simulink model "model"  (R2014a)
(part 6 of 6)

  _CN_235143897_220000_CN_21239912_220000/LConn1 -- T_235143897__SP_AusNet_Brooklyn_Terminal_Station/LConn1 -- _CN_235143897_220000_CN_384601555_220000/LConn1 -- _CN_235143897_220000_CN_243897689_220000/LConn1
  _CN_235143897_220000_CN_21239912_220000/LConn2 -- T_235143897__SP_AusNet_Brooklyn_Terminal_Station/LConn2 -- _CN_235143897_220000_CN_384601555_220000/LConn2 -- _CN_235143897_220000_CN_243897689_220000/LConn2
  _CN_235143897_220000_CN_21239912_220000/LConn3 -- T_235143897__SP_AusNet_Brooklyn_Terminal_Station/LConn3 -- _CN_235143897_220000_CN_384601555_220000/LConn3 -- _CN_235143897_220000_CN_243897689_220000/LConn3 -- bus266/LConn1
  _CN_235143897_220000_CN_21239912_220000/RConn1 -- T_21239912__AusNet_Keilor_Terminal_Station/RConn1 -- _CN_23718970_220000_CN_21239912_220000/LConn1 -- _CN_21239912_220000_CN_208198646_220000/LConn1 -- L_21239912/LConn1 -- _CN_244141232_220000_CN_21239912_220000/LConn1
  _CN_235143897_220000_CN_21239912_220000/RConn2 -- T_21239912__AusNet_Keilor_Terminal_Station/RConn2 -- _CN_23718970_220000_CN_21239912_220000/LConn2 -- _CN_21239912_220000_CN_208198646_220000/LConn2 -- L_21239912/LConn2 -- _CN_244141232_220000_CN_21239912_220000/LConn2
  _CN_235143897_220000_CN_21239912_220000/RConn3 -- T_21239912__AusNet_Keilor_Terminal_Station/RConn3 -- _CN_23718970_220000_CN_21239912_220000/LConn3 -- _CN_21239912_220000_CN_208198646_220000/LConn3 -- L_21239912/LConn3 -- bus267/LConn1 -- _CN_244141232_220000_CN_21239912_220000/LConn3
  _CN_235143897_220000_CN_384601555_220000/RConn1 -- T_384601555__AusNet_Fishermans_Bend_Terminal_Station/LConn1 -- _CN_384601555_220000_CN_208198646_220000/LConn1
  _CN_235143897_220000_CN_384601555_220000/RConn2 -- T_384601555__AusNet_Fishermans_Bend_Terminal_Station/LConn2 -- _CN_384601555_220000_CN_208198646_220000/LConn2
  _CN_235143897_220000_CN_384601555_220000/RConn3 -- T_384601555__AusNet_Fishermans_Bend_Terminal_Station/LConn3 -- _CN_384601555_220000_CN_208198646_220000/LConn3 -- bus268/LConn1
  G_243897689_Ecogen_Newport_Power_Station/RConn1 -- _CN_235143897_220000_CN_243897689_220000/RConn1
  G_243897689_Ecogen_Newport_Power_Station/RConn2 -- _CN_235143897_220000_CN_243897689_220000/RConn2
  _CN_235143897_220000_CN_243897689_220000/RConn3 -- G_243897689_Ecogen_Newport_Power_Station/RConn3 -- bus269/LConn1
  T_23298443__/LConn1 -- _CN_23298443_220000_CN_87324834_220000/LConn1
  T_23298443__/LConn2 -- _CN_23298443_220000_CN_87324834_220000/LConn2
  _CN_23298443_220000_CN_87324834_220000/LConn3 -- T_23298443__/LConn3 -- bus270/LConn1
  _CN_23298443_220000_CN_87324834_220000/RConn1 -- G_87324834_Liapootah_Power_Station/RConn1 -- _CN_87325631_220000_CN_87324834_220000/LConn1
  _CN_23298443_220000_CN_87324834_220000/RConn2 -- G_87324834_Liapootah_Power_Station/RConn2 -- _CN_87325631_220000_CN_87324834_220000/LConn2
  _CN_23298443_220000_CN_87324834_220000/RConn3 -- G_87324834_Liapootah_Power_Station/RConn3 -- _CN_87325631_220000_CN_87324834_220000/LConn3 -- bus271/LConn1
  T_167791635__Burnie_Substation/LConn1 -- _CN_167791635_220000_CN_88191017_220000/LConn1
  T_167791635__Burnie_Substation/LConn2 -- _CN_167791635_220000_CN_88191017_220000/LConn2
  _CN_167791635_220000_CN_88191017_220000/LConn3 -- T_167791635__Burnie_Substation/LConn3 -- bus272/LConn1
  _CN_167791635_220000_CN_88191017_220000/RConn1 -- T_88191017__/LConn1 -- _CN_88191017_220000_CN_174441055_220000/RConn1
  _CN_167791635_220000_CN_88191017_220000/RConn2 -- T_88191017__/LConn2 -- _CN_88191017_220000_CN_174441055_220000/RConn2
  _CN_167791635_220000_CN_88191017_220000/RConn3 -- T_88191017__/LConn3 -- _CN_88191017_220000_CN_174441055_220000/RConn3 -- bus273/LConn1
  _CN_24054804_220000_CN_28225387_220000/LConn1 -- T_24054804__SP_AusNet_Rowville_Terminal_Station/RConn1 -- _CN_24054804_220000_CN_30837800_220000/LConn1 -- _CN_24054804_220000_CN_134534513_220000/LConn1 -- L_24054804/LConn1 -- _CN_24054804_220000_CN_239972088_220000/LConn1
  _CN_24054804_220000_CN_28225387_220000/LConn2 -- T_24054804__SP_AusNet_Rowville_Terminal_Station/RConn2 -- _CN_24054804_220000_CN_30837800_220000/LConn2 -- _CN_24054804_220000_CN_134534513_220000/LConn2 -- L_24054804/LConn2 -- _CN_24054804_220000_CN_239972088_220000/LConn2
  _CN_24054804_220000_CN_28225387_220000/LConn3 -- T_24054804__SP_AusNet_Rowville_Terminal_Station/RConn3 -- _CN_24054804_220000_CN_30837800_220000/LConn3 -- _CN_24054804_220000_CN_134534513_220000/LConn3 -- L_24054804/LConn3 -- bus274/LConn1 -- _CN_24054804_220000_CN_239972088_220000/LConn3
  T_28225387__SP_AusNet_Malvern_Terminal_Station/LConn1 -- _CN_24054804_220000_CN_28225387_220000/RConn1
  T_28225387__SP_AusNet_Malvern_Terminal_Station/LConn2 -- _CN_24054804_220000_CN_28225387_220000/RConn2
  _CN_24054804_220000_CN_28225387_220000/RConn3 -- T_28225387__SP_AusNet_Malvern_Terminal_Station/LConn3 -- bus275/LConn1
  _CN_24054804_220000_CN_239972088_220000/RConn1 -- T_239972088__SP_AusNet_Rowville_East_Terminal_Station/LConn1 -- _CN_48955336_220000_CN_239972088_220000/LConn1
  _CN_24054804_220000_CN_239972088_220000/RConn2 -- T_239972088__SP_AusNet_Rowville_East_Terminal_Station/LConn2 -- _CN_48955336_220000_CN_239972088_220000/LConn2
  _CN_24054804_220000_CN_239972088_220000/RConn3 -- T_239972088__SP_AusNet_Rowville_East_Terminal_Station/LConn3 -- _CN_48955336_220000_CN_239972088_220000/LConn3 -- bus276/LConn1
  _CN_24054804_220000_CN_30837800_220000/RConn1 -- T_30837800__SP_AusNet_Richmond_Terminal_Station/LConn1 -- _CN_30837800_220000_CN_41098451_220000/LConn1
  _CN_24054804_220000_CN_30837800_220000/RConn2 -- T_30837800__SP_AusNet_Richmond_Terminal_Station/LConn2 -- _CN_30837800_220000_CN_41098451_220000/LConn2
  _CN_24054804_220000_CN_30837800_220000/RConn3 -- T_30837800__SP_AusNet_Richmond_Terminal_Station/LConn3 -- _CN_30837800_220000_CN_41098451_220000/LConn3 -- bus277/LConn1
  _CN_24054804_220000_CN_134534513_220000/RConn1 -- T_134534513__AusNet_Springvale_Terminal_Station/LConn1 -- _CN_28917073_220000_CN_134534513_220000/LConn1
  _CN_24054804_220000_CN_134534513_220000/RConn2 -- T_134534513__AusNet_Springvale_Terminal_Station/LConn2 -- _CN_28917073_220000_CN_134534513_220000/LConn2
  _CN_24054804_220000_CN_134534513_220000/RConn3 -- T_134534513__AusNet_Springvale_Terminal_Station/LConn3 -- _CN_28917073_220000_CN_134534513_220000/LConn3 -- bus278/LConn1
  T_169794711__/LConn1 -- _CN_169794711_220000_CN_172740336_220000/LConn1
  T_169794711__/LConn2 -- _CN_169794711_220000_CN_172740336_220000/LConn2
  _CN_169794711_220000_CN_172740336_220000/LConn3 -- T_169794711__/LConn3 -- bus279/LConn1
  T_172740336__/LConn1 -- _CN_169794711_220000_CN_172740336_220000/RConn1
  T_172740336__/LConn2 -- _CN_169794711_220000_CN_172740336_220000/RConn2
  _CN_169794711_220000_CN_172740336_220000/RConn3 -- T_172740336__/LConn3 -- bus280/LConn1
  _CN_30837800_220000_CN_41098451_220000/RConn1 -- T_41098451_220000;22000_SP_AusNet_Brunswick_Terminal_Station/LConn1 -- _CN_23718970_220000_CN_41098451_220000/LConn1
  _CN_30837800_220000_CN_41098451_220000/RConn2 -- T_41098451_220000;22000_SP_AusNet_Brunswick_Terminal_Station/LConn2 -- _CN_23718970_220000_CN_41098451_220000/LConn2
  _CN_30837800_220000_CN_41098451_220000/RConn3 -- T_41098451_220000;22000_SP_AusNet_Brunswick_Terminal_Station/LConn3 -- _CN_23718970_220000_CN_41098451_220000/LConn3 -- bus281/LConn1
  T_24577195__SP_AusNet_Ringwood_Terminal_Station/LConn1 -- _CN_24577195_220000_CN_23718111_220000/LConn1
  T_24577195__SP_AusNet_Ringwood_Terminal_Station/LConn2 -- _CN_24577195_220000_CN_23718111_220000/LConn2
  _CN_24577195_220000_CN_23718111_220000/LConn3 -- T_24577195__SP_AusNet_Ringwood_Terminal_Station/LConn3 -- bus282/LConn1
  _CN_24577195_220000_CN_23718111_220000/RConn1 -- T_23718111__SP_AusNet_Templestowe_Terminal_Station/LConn1 -- _CN_23718970_220000_CN_23718111_220000/LConn1
  _CN_24577195_220000_CN_23718111_220000/RConn2 -- T_23718111__SP_AusNet_Templestowe_Terminal_Station/LConn2 -- _CN_23718970_220000_CN_23718111_220000/LConn2
  _CN_24577195_220000_CN_23718111_220000/RConn3 -- T_23718111__SP_AusNet_Templestowe_Terminal_Station/LConn3 -- _CN_23718970_220000_CN_23718111_220000/LConn3 -- bus283/LConn1
  _CN_244141232_220000_CN_21239912_220000/RConn1 -- T_244141232__SP_AusNet_Geelong_Terminal_Station/LConn1 -- _CN_244141232_220000_CN_49455810_220000/RConn1
  _CN_244141232_220000_CN_21239912_220000/RConn2 -- T_244141232__SP_AusNet_Geelong_Terminal_Station/LConn2 -- _CN_244141232_220000_CN_49455810_220000/RConn2
  _CN_244141232_220000_CN_21239912_220000/RConn3 -- T_244141232__SP_AusNet_Geelong_Terminal_Station/LConn3 -- _CN_244141232_220000_CN_49455810_220000/RConn3 -- bus284/LConn1
  T_169793928__/LConn1 -- _CN_169793928_220000_CN_239996090_220000/LConn1
  T_169793928__/LConn2 -- _CN_169793928_220000_CN_239996090_220000/LConn2
  _CN_169793928_220000_CN_239996090_220000/LConn3 -- T_169793928__/LConn3 -- bus285/LConn1
  T_239996090__SP_AusNet_Wemen_Terminal_Station/LConn1 -- _CN_169793928_220000_CN_239996090_220000/RConn1
  T_239996090__SP_AusNet_Wemen_Terminal_Station/LConn2 -- _CN_169793928_220000_CN_239996090_220000/RConn2
  _CN_169793928_220000_CN_239996090_220000/RConn3 -- T_239996090__SP_AusNet_Wemen_Terminal_Station/LConn3 -- bus286/LConn1
  _CN_56234037_220000_CN_64943050_220000/RConn1 -- T_64943050__SP_AusNet_South_Morang_Terminal_Station/LConn1 -- _CN_23718970_220000_CN_64943050_220000/LConn1
  _CN_56234037_220000_CN_64943050_220000/RConn2 -- T_64943050__SP_AusNet_South_Morang_Terminal_Station/LConn2 -- _CN_23718970_220000_CN_64943050_220000/LConn2
  _CN_56234037_220000_CN_64943050_220000/RConn3 -- T_64943050__SP_AusNet_South_Morang_Terminal_Station/LConn3 -- _CN_23718970_220000_CN_64943050_220000/LConn3 -- bus287/LConn1
  _CN_286063160_220000_CN_205163985_220000/RConn1 -- T_205163985__Glenrowan_Terminal_Station/LConn1 -- _CN_174893662_220000_CN_205163985_220000/LConn1
  _CN_286063160_220000_CN_205163985_220000/RConn2 -- T_205163985__Glenrowan_Terminal_Station/LConn2 -- _CN_174893662_220000_CN_205163985_220000/LConn2
  _CN_286063160_220000_CN_205163985_220000/RConn3 -- T_205163985__Glenrowan_Terminal_Station/LConn3 -- _CN_174893662_220000_CN_205163985_220000/LConn3 -- bus288/LConn1
  _CN_23718970_220000_CN_21239912_220000/RConn1 -- T_23718970__SP_AusNet_Thomastown_Terminal_Station/LConn1 -- _CN_23718970_220000_CN_64943050_220000/RConn1 -- _CN_23718970_220000_CN_23718111_220000/RConn1 -- _CN_23718970_220000_CN_41098451_220000/RConn1
  _CN_23718970_220000_CN_21239912_220000/RConn2 -- T_23718970__SP_AusNet_Thomastown_Terminal_Station/LConn2 -- _CN_23718970_220000_CN_64943050_220000/RConn2 -- _CN_23718970_220000_CN_23718111_220000/RConn2 -- _CN_23718970_220000_CN_41098451_220000/RConn2
  _CN_23718970_220000_CN_21239912_220000/RConn3 -- T_23718970__SP_AusNet_Thomastown_Terminal_Station/LConn3 -- _CN_23718970_220000_CN_64943050_220000/RConn3 -- _CN_23718970_220000_CN_23718111_220000/RConn3 -- _CN_23718970_220000_CN_41098451_220000/RConn3 -- bus289/LConn1
  _CN_87325631_220000_CN_87324834_220000/RConn1 -- T_87325631__/LConn1 -- _CN_87325631_220000_CN_87327101_220000/LConn1
  _CN_87325631_220000_CN_87324834_220000/RConn2 -- T_87325631__/LConn2 -- _CN_87325631_220000_CN_87327101_220000/LConn2
  _CN_87325631_220000_CN_87324834_220000/RConn3 -- T_87325631__/LConn3 -- _CN_87325631_220000_CN_87327101_220000/LConn3 -- bus290/LConn1
  G_87327101_Catagunya_Power_Station/RConn1 -- _CN_87325631_220000_CN_87327101_220000/RConn1
  G_87327101_Catagunya_Power_Station/RConn2 -- _CN_87325631_220000_CN_87327101_220000/RConn2
  _CN_87325631_220000_CN_87327101_220000/RConn3 -- G_87327101_Catagunya_Power_Station/RConn3 -- bus291/LConn1
  _CN_48955336_220000_CN_239972088_220000/RConn1 -- T_48955336__SP_AusNet_Cranbourne_Terminal_Station/RConn1 -- L_48955336/LConn1
  _CN_48955336_220000_CN_239972088_220000/RConn2 -- T_48955336__SP_AusNet_Cranbourne_Terminal_Station/RConn2 -- L_48955336/LConn2
  _CN_48955336_220000_CN_239972088_220000/RConn3 -- T_48955336__SP_AusNet_Cranbourne_Terminal_Station/RConn3 -- L_48955336/LConn3 -- bus292/LConn1
  _CN_223942734_220000_CN_223940475_220000/RConn1 -- T_223940475__/LConn1 -- _CN_223939702_220000_CN_223940475_220000/LConn1
  _CN_223942734_220000_CN_223940475_220000/RConn2 -- T_223940475__/LConn2 -- _CN_223939702_220000_CN_223940475_220000/LConn2
  _CN_223942734_220000_CN_223940475_220000/RConn3 -- T_223940475__/LConn3 -- _CN_223939702_220000_CN_223940475_220000/LConn3 -- bus293/LConn1
  T_28917073__SP_AusNet_Heatherton_Terminal_Station/LConn1 -- _CN_28917073_220000_CN_134534513_220000/RConn1
  T_28917073__SP_AusNet_Heatherton_Terminal_Station/LConn2 -- _CN_28917073_220000_CN_134534513_220000/RConn2
  _CN_28917073_220000_CN_134534513_220000/RConn3 -- T_28917073__SP_AusNet_Heatherton_Terminal_Station/LConn3 -- bus294/LConn1
  T_218402190__/LConn1 -- _CN_218402190_220000_CN_229759860_220000/LConn1
  T_218402190__/LConn2 -- _CN_218402190_220000_CN_229759860_220000/LConn2
  _CN_218402190_220000_CN_229759860_220000/LConn3 -- T_218402190__/LConn3 -- bus295/LConn1
  T_229759860__/LConn1 -- _CN_218402190_220000_CN_229759860_220000/RConn1
  T_229759860__/LConn2 -- _CN_218402190_220000_CN_229759860_220000/RConn2
  _CN_218402190_220000_CN_229759860_220000/RConn3 -- T_229759860__/LConn3 -- bus296/LConn1
  _CN_174893662_220000_CN_173566563_220000/LConn1 -- T_174893662__Shepparton_Terminal_Station/LConn1 -- _CN_174893662_220000_CN_205163985_220000/RConn1
  _CN_174893662_220000_CN_173566563_220000/LConn2 -- T_174893662__Shepparton_Terminal_Station/LConn2 -- _CN_174893662_220000_CN_205163985_220000/RConn2
  _CN_174893662_220000_CN_173566563_220000/LConn3 -- T_174893662__Shepparton_Terminal_Station/LConn3 -- _CN_174893662_220000_CN_205163985_220000/RConn3 -- bus297/LConn1
  T_173566563__AusNet_Foxterville_Terminal_Station/LConn1 -- _CN_174893662_220000_CN_173566563_220000/RConn1
  T_173566563__AusNet_Foxterville_Terminal_Station/LConn2 -- _CN_174893662_220000_CN_173566563_220000/RConn2
  _CN_174893662_220000_CN_173566563_220000/RConn3 -- T_173566563__AusNet_Foxterville_Terminal_Station/LConn3 -- bus298/LConn1
  _CN_21239912_220000_CN_208198646_220000/RConn1 -- T_208198646__AusNet_West_Melbourne_Terminal_Station/LConn1 -- _CN_384601555_220000_CN_208198646_220000/RConn1
  _CN_21239912_220000_CN_208198646_220000/RConn2 -- T_208198646__AusNet_West_Melbourne_Terminal_Station/LConn2 -- _CN_384601555_220000_CN_208198646_220000/RConn2
  _CN_21239912_220000_CN_208198646_220000/RConn3 -- T_208198646__AusNet_West_Melbourne_Terminal_Station/LConn3 -- _CN_384601555_220000_CN_208198646_220000/RConn3 -- bus299/LConn1
  T_223939702__/LConn1 -- _CN_223939702_220000_CN_223940475_220000/RConn1
  T_223939702__/LConn2 -- _CN_223939702_220000_CN_223940475_220000/RConn2
  _CN_223939702_220000_CN_223940475_220000/RConn3 -- T_223939702__/LConn3 -- bus300/LConn1
  T_196363948__/LConn1 -- _CN_196363948_275000_CN_189021414_275000/LConn1
  T_196363948__/LConn2 -- _CN_196363948_275000_CN_189021414_275000/LConn2
  _CN_196363948_275000_CN_189021414_275000/LConn3 -- T_196363948__/LConn3 -- bus301/LConn1
  _CN_196363948_275000_CN_189021414_275000/RConn1 -- T_189021414__/LConn1 -- _CN_173700961_275000_CN_189021414_275000/LConn1
  _CN_196363948_275000_CN_189021414_275000/RConn2 -- T_189021414__/LConn2 -- _CN_173700961_275000_CN_189021414_275000/LConn2
  _CN_196363948_275000_CN_189021414_275000/RConn3 -- T_189021414__/LConn3 -- _CN_173700961_275000_CN_189021414_275000/LConn3 -- bus302/LConn1
  _CN_172587651_275000_CN_172878761_275000/LConn1 -- T_172587651__Greenbank_Substation/LConn1 -- _CN_172587651_275000_CN_173222725_275000/LConn1 -- _CN_172587651_275000_CN_46099414_275000/LConn1 -- _CN_172587651_275000_CN_176443359_275000/LConn1 -- _CN_172587651_275000_CN_95612087_275000/LConn1 -- _CN_172587651_275000_CN_45020488_275000/LConn1
  _CN_172587651_275000_CN_172878761_275000/LConn2 -- T_172587651__Greenbank_Substation/LConn2 -- _CN_172587651_275000_CN_173222725_275000/LConn2 -- _CN_172587651_275000_CN_46099414_275000/LConn2 -- _CN_172587651_275000_CN_176443359_275000/LConn2 -- _CN_172587651_275000_CN_95612087_275000/LConn2 -- _CN_172587651_275000_CN_45020488_275000/LConn2
  _CN_172587651_275000_CN_172878761_275000/LConn3 -- T_172587651__Greenbank_Substation/LConn3 -- _CN_172587651_275000_CN_173222725_275000/LConn3 -- _CN_172587651_275000_CN_46099414_275000/LConn3 -- bus303/LConn1 -- _CN_172587651_275000_CN_176443359_275000/LConn3 -- _CN_172587651_275000_CN_95612087_275000/LConn3 -- _CN_172587651_275000_CN_45020488_275000/LConn3
  _CN_172587651_275000_CN_172878761_275000/RConn1 -- T_172878761__Middle_Ridge_Substation/LConn1 -- _CN_170709510_275000_CN_172878761_275000/LConn1
  _CN_172587651_275000_CN_172878761_275000/RConn2 -- T_172878761__Middle_Ridge_Substation/LConn2 -- _CN_170709510_275000_CN_172878761_275000/LConn2
  _CN_172587651_275000_CN_172878761_275000/RConn3 -- T_172878761__Middle_Ridge_Substation/LConn3 -- _CN_170709510_275000_CN_172878761_275000/LConn3 -- bus304/LConn1
  T_95612087__/LConn1 -- _CN_172587651_275000_CN_95612087_275000/RConn1
  T_95612087__/LConn2 -- _CN_172587651_275000_CN_95612087_275000/RConn2
  _CN_172587651_275000_CN_95612087_275000/RConn3 -- T_95612087__/LConn3 -- bus305/LConn1
  T_45020488__Mudgeeraba_Substation/LConn1 -- _CN_172587651_275000_CN_45020488_275000/RConn1
  T_45020488__Mudgeeraba_Substation/LConn2 -- _CN_172587651_275000_CN_45020488_275000/RConn2
  _CN_172587651_275000_CN_45020488_275000/RConn3 -- T_45020488__Mudgeeraba_Substation/LConn3 -- bus306/LConn1
  T_176443359__Bundamba_Substation/LConn1 -- _CN_172587651_275000_CN_176443359_275000/RConn1
  T_176443359__Bundamba_Substation/LConn2 -- _CN_172587651_275000_CN_176443359_275000/RConn2
  _CN_172587651_275000_CN_176443359_275000/RConn3 -- T_176443359__Bundamba_Substation/LConn3 -- bus307/LConn1
  T_173222725__/LConn1 -- _CN_172587651_275000_CN_173222725_275000/RConn1
  T_173222725__/LConn2 -- _CN_172587651_275000_CN_173222725_275000/RConn2
  _CN_172587651_275000_CN_173222725_275000/RConn3 -- T_173222725__/LConn3 -- bus308/LConn1
  T_46099414__Loganlea_Substation/LConn1 -- _CN_172587651_275000_CN_46099414_275000/RConn1
  T_46099414__Loganlea_Substation/LConn2 -- _CN_172587651_275000_CN_46099414_275000/RConn2
  _CN_172587651_275000_CN_46099414_275000/RConn3 -- T_46099414__Loganlea_Substation/LConn3 -- bus309/LConn1
  _CN_170709510_275000_CN_170842253_275000/LConn1 -- T_170709510__/LConn1 -- _CN_170709510_275000_CN_170832455_275000/LConn1 -- _CN_170709510_275000_CN_153737699_275000/LConn1 -- _CN_170709510_275000_CN_19384720_275000/LConn1 -- _CN_170709510_275000_CN_172878761_275000/RConn1
  _CN_170709510_275000_CN_170842253_275000/LConn2 -- T_170709510__/LConn2 -- _CN_170709510_275000_CN_170832455_275000/LConn2 -- _CN_170709510_275000_CN_153737699_275000/LConn2 -- _CN_170709510_275000_CN_19384720_275000/LConn2 -- _CN_170709510_275000_CN_172878761_275000/RConn2
  _CN_170709510_275000_CN_170842253_275000/LConn3 -- T_170709510__/LConn3 -- _CN_170709510_275000_CN_170832455_275000/LConn3 -- _CN_170709510_275000_CN_153737699_275000/LConn3 -- _CN_170709510_275000_CN_19384720_275000/LConn3 -- bus310/LConn1 -- _CN_170709510_275000_CN_172878761_275000/RConn3
  _CN_170709510_275000_CN_170842253_275000/RConn1 -- T_170842253__Braemar/RConn1 -- L_170842253/LConn1
  _CN_170709510_275000_CN_170842253_275000/RConn2 -- T_170842253__Braemar/RConn2 -- L_170842253/LConn2
  _CN_170709510_275000_CN_170842253_275000/RConn3 -- T_170842253__Braemar/RConn3 -- L_170842253/LConn3 -- bus311/LConn1
  _CN_170709510_275000_CN_170832455_275000/RConn1 -- T_170832455__/LConn1 -- Swanbank___South_Pine_CN_19384720_275000_CN_170832455_275000/LConn1 -- _CN_170832455_275000_CN_173223683_275000/LConn1 -- _CN_170832455_275000_CN_153737699_275000/LConn1 -- _CN_170832455_275000_CN_19380255_110000/RConn1
  _CN_170709510_275000_CN_170832455_275000/RConn2 -- T_170832455__/LConn2 -- Swanbank___South_Pine_CN_19384720_275000_CN_170832455_275000/LConn2 -- _CN_170832455_275000_CN_173223683_275000/LConn2 -- _CN_170832455_275000_CN_153737699_275000/LConn2 -- _CN_170832455_275000_CN_19380255_110000/RConn2
  _CN_170709510_275000_CN_170832455_275000/RConn3 -- T_170832455__/LConn3 -- Swanbank___South_Pine_CN_19384720_275000_CN_170832455_275000/LConn3 -- _CN_170832455_275000_CN_173223683_275000/LConn3 -- _CN_170832455_275000_CN_153737699_275000/LConn3 -- _CN_170832455_275000_CN_19380255_110000/RConn3 -- bus312/LConn1
  _CN_170709510_275000_CN_153737699_275000/RConn1 -- T_153737699__/LConn1 -- _CN_170832455_275000_CN_153737699_275000/RConn1
  _CN_170709510_275000_CN_153737699_275000/RConn2 -- T_153737699__/LConn2 -- _CN_170832455_275000_CN_153737699_275000/RConn2
  _CN_170709510_275000_CN_153737699_275000/RConn3 -- T_153737699__/LConn3 -- _CN_170832455_275000_CN_153737699_275000/RConn3 -- bus313/LConn1
  _CN_170709510_275000_CN_19384720_275000/RConn1 -- T_19384720__South_Pine_Substation/LConn1 -- _CN_19384720_275000_CN_170990862_275000/LConn1 -- Swanbank___South_Pine_CN_19384720_275000_CN_170832455_275000/RConn1
  _CN_170709510_275000_CN_19384720_275000/RConn2 -- T_19384720__South_Pine_Substation/LConn2 -- _CN_19384720_275000_CN_170990862_275000/LConn2 -- Swanbank___South_Pine_CN_19384720_275000_CN_170832455_275000/RConn2
  _CN_170709510_275000_CN_19384720_275000/RConn3 -- T_19384720__South_Pine_Substation/LConn3 -- _CN_19384720_275000_CN_170990862_275000/LConn3 -- Swanbank___South_Pine_CN_19384720_275000_CN_170832455_275000/RConn3 -- bus314/LConn1
  _CN_171170697_275000_CN_171728751_275000/LConn1 -- T_171170697__/LConn1 -- _CN_171170697_275000_CN_432510474_275000/LConn1 -- _CN_171170697_275000_CN_119995150_275000/LConn1
  _CN_171170697_275000_CN_171728751_275000/LConn2 -- T_171170697__/LConn2 -- _CN_171170697_275000_CN_432510474_275000/LConn2 -- _CN_171170697_275000_CN_119995150_275000/LConn2
  _CN_171170697_275000_CN_171728751_275000/LConn3 -- T_171170697__/LConn3 -- _CN_171170697_275000_CN_432510474_275000/LConn3 -- _CN_171170697_275000_CN_119995150_275000/LConn3 -- bus315/LConn1
  _CN_171170697_275000_CN_171728751_275000/RConn1 -- T_171728751__Gin_Gin_terminal_station/LConn1 -- _CN_432510474_275000_CN_171728751_275000/LConn1 -- _CN_170990862_275000_CN_171728751_275000/LConn1 -- _CN_171002668_275000_CN_171728751_275000/LConn1
  _CN_171170697_275000_CN_171728751_275000/RConn2 -- T_171728751__Gin_Gin_terminal_station/LConn2 -- _CN_432510474_275000_CN_171728751_275000/LConn2 -- _CN_170990862_275000_CN_171728751_275000/LConn2 -- _CN_171002668_275000_CN_171728751_275000/LConn2
  _CN_171170697_275000_CN_171728751_275000/RConn3 -- T_171728751__Gin_Gin_terminal_station/LConn3 -- _CN_432510474_275000_CN_171728751_275000/LConn3 -- _CN_170990862_275000_CN_171728751_275000/LConn3 -- _CN_171002668_275000_CN_171728751_275000/LConn3 -- bus316/LConn1
  _CN_171170697_275000_CN_432510474_275000/RConn1 -- T_432510474__Calliope_River_Substation/LConn1 -- _CN_432510474_275000_CN_54674751_275000/LConn1 -- _CN_432510474_275000_CN_171486427_275000/LConn1 -- _CN_432510474_275000_CN_171728751_275000/RConn1
  _CN_171170697_275000_CN_432510474_275000/RConn2 -- T_432510474__Calliope_River_Substation/LConn2 -- _CN_432510474_275000_CN_54674751_275000/LConn2 -- _CN_432510474_275000_CN_171486427_275000/LConn2 -- _CN_432510474_275000_CN_171728751_275000/RConn2
  _CN_171170697_275000_CN_432510474_275000/RConn3 -- T_432510474__Calliope_River_Substation/LConn3 -- _CN_432510474_275000_CN_54674751_275000/LConn3 -- bus317/LConn1 -- _CN_432510474_275000_CN_171486427_275000/LConn3 -- _CN_432510474_275000_CN_171728751_275000/RConn3
  T_119995150__Callide_Switch_Yard/LConn1 -- _CN_171170697_275000_CN_119995150_275000/RConn1
  T_119995150__Callide_Switch_Yard/LConn2 -- _CN_171170697_275000_CN_119995150_275000/RConn2
  _CN_171170697_275000_CN_119995150_275000/RConn3 -- T_119995150__Callide_Switch_Yard/LConn3 -- bus318/LConn1
  _CN_432510474_275000_CN_171486427_275000/RConn1 -- T_171486427__/LConn1 -- _CN_171486427_275000_CN_121646942_275000/LConn1
  _CN_432510474_275000_CN_171486427_275000/RConn2 -- T_171486427__/LConn2 -- _CN_171486427_275000_CN_121646942_275000/LConn2
  _CN_432510474_275000_CN_171486427_275000/RConn3 -- T_171486427__/LConn3 -- _CN_171486427_275000_CN_121646942_275000/LConn3 -- bus319/LConn1
  T_54674751__Gladstone_Power_Station_Sub_Station/LConn1 -- _CN_432510474_275000_CN_54674751_275000/RConn1
  T_54674751__Gladstone_Power_Station_Sub_Station/LConn2 -- _CN_432510474_275000_CN_54674751_275000/RConn2
  _CN_432510474_275000_CN_54674751_275000/RConn3 -- T_54674751__Gladstone_Power_Station_Sub_Station/LConn3 -- bus320/LConn1
  _CN_19384720_275000_CN_170990862_275000/RConn1 -- T_170990862__/LConn1 -- _CN_170990862_275000_CN_171002668_275000/LConn1 -- _CN_170990862_275000_CN_171728751_275000/RConn1
  _CN_19384720_275000_CN_170990862_275000/RConn2 -- T_170990862__/LConn2 -- _CN_170990862_275000_CN_171002668_275000/LConn2 -- _CN_170990862_275000_CN_171728751_275000/RConn2
  _CN_19384720_275000_CN_170990862_275000/RConn3 -- T_170990862__/LConn3 -- _CN_170990862_275000_CN_171002668_275000/LConn3 -- _CN_170990862_275000_CN_171728751_275000/RConn3 -- bus321/LConn1
  _CN_170990862_275000_CN_171002668_275000/RConn1 -- T_171002668__/LConn1 -- _CN_171002668_275000_CN_171728751_275000/RConn1
  _CN_170990862_275000_CN_171002668_275000/RConn2 -- T_171002668__/LConn2 -- _CN_171002668_275000_CN_171728751_275000/RConn2
  _CN_170990862_275000_CN_171002668_275000/RConn3 -- T_171002668__/LConn3 -- _CN_171002668_275000_CN_171728751_275000/RConn3 -- bus322/LConn1
  _CN_172715843_275000_CN_172715454_275000/LConn1 -- T_172715843__Electranet_Northfield_Substation/LConn1 -- _CN_172715843_275000_CN_172714953_275000/LConn1
  _CN_172715843_275000_CN_172715454_275000/LConn2 -- T_172715843__Electranet_Northfield_Substation/LConn2 -- _CN_172715843_275000_CN_172714953_275000/LConn2
  _CN_172715843_275000_CN_172715454_275000/LConn3 -- T_172715843__Electranet_Northfield_Substation/LConn3 -- _CN_172715843_275000_CN_172714953_275000/LConn3 -- bus323/LConn1
  G_172715454_Dry_Creek_Power_Station/RConn1 -- _CN_172715843_275000_CN_172715454_275000/RConn1
  G_172715454_Dry_Creek_Power_Station/RConn2 -- _CN_172715843_275000_CN_172715454_275000/RConn2
  _CN_172715843_275000_CN_172715454_275000/RConn3 -- G_172715454_Dry_Creek_Power_Station/RConn3 -- bus324/LConn1
  _CN_172715843_275000_CN_172714953_275000/RConn1 -- G_172714953_Torrens_Island_Power_Station/RConn1 -- _CN_172714955_275000_CN_172714953_275000/LConn1
  _CN_172715843_275000_CN_172714953_275000/RConn2 -- G_172714953_Torrens_Island_Power_Station/RConn2 -- _CN_172714955_275000_CN_172714953_275000/LConn2
  _CN_172715843_275000_CN_172714953_275000/RConn3 -- G_172714953_Torrens_Island_Power_Station/RConn3 -- _CN_172714955_275000_CN_172714953_275000/LConn3 -- bus325/LConn1
  T_26230300__Belmont_Substation/LConn1 -- _CN_26230300_275000_CN_44418650_275000/LConn1
  T_26230300__Belmont_Substation/LConn2 -- _CN_26230300_275000_CN_44418650_275000/LConn2
  _CN_26230300_275000_CN_44418650_275000/LConn3 -- T_26230300__Belmont_Substation/LConn3 -- bus326/LConn1
  T_44418650__/LConn1 -- _CN_26230300_275000_CN_44418650_275000/RConn1
  T_44418650__/LConn2 -- _CN_26230300_275000_CN_44418650_275000/RConn2
  _CN_26230300_275000_CN_44418650_275000/RConn3 -- T_44418650__/LConn3 -- bus327/LConn1
  T_169673123__Heywood/LConn1 -- _CN_169673123_275000_CN_164675939_275000/LConn1
  T_169673123__Heywood/LConn2 -- _CN_169673123_275000_CN_164675939_275000/LConn2
  _CN_169673123_275000_CN_164675939_275000/LConn3 -- T_169673123__Heywood/LConn3 -- bus328/LConn1
  _CN_169673123_275000_CN_164675939_275000/RConn1 -- T_164675939__ElectraNet_South_East_Substation/LConn1 -- _CN_164675939_275000_CN_75514732_275000/LConn1
  _CN_169673123_275000_CN_164675939_275000/RConn2 -- T_164675939__ElectraNet_South_East_Substation/LConn2 -- _CN_164675939_275000_CN_75514732_275000/LConn2
  _CN_169673123_275000_CN_164675939_275000/RConn3 -- T_164675939__ElectraNet_South_East_Substation/LConn3 -- _CN_164675939_275000_CN_75514732_275000/LConn3 -- bus329/LConn1
  _CN_224209320_275000_CN_172362099_275000/LConn1 -- T_224209320__/LConn1 -- _CN_224209320_275000_CN_75514732_275000/LConn1 -- _CN_224209320_275000_CN_172364007_275000/LConn1
  _CN_224209320_275000_CN_172362099_275000/LConn2 -- T_224209320__/LConn2 -- _CN_224209320_275000_CN_75514732_275000/LConn2 -- _CN_224209320_275000_CN_172364007_275000/LConn2
  _CN_224209320_275000_CN_172362099_275000/LConn3 -- T_224209320__/LConn3 -- _CN_224209320_275000_CN_75514732_275000/LConn3 -- _CN_224209320_275000_CN_172364007_275000/LConn3 -- bus330/LConn1
  _CN_224209320_275000_CN_172362099_275000/RConn1 -- T_172362099__/LConn1 -- _CN_170058930_275000_CN_172362099_275000/LConn1 -- _CN_172364006_275000_CN_172362099_275000/LConn1 -- _CN_172364007_275000_CN_172362099_275000/LConn1
  _CN_224209320_275000_CN_172362099_275000/RConn2 -- T_172362099__/LConn2 -- _CN_170058930_275000_CN_172362099_275000/LConn2 -- _CN_172364006_275000_CN_172362099_275000/LConn2 -- _CN_172364007_275000_CN_172362099_275000/LConn2
  _CN_224209320_275000_CN_172362099_275000/RConn3 -- T_172362099__/LConn3 -- _CN_170058930_275000_CN_172362099_275000/LConn3 -- _CN_172364006_275000_CN_172362099_275000/LConn3 -- _CN_172364007_275000_CN_172362099_275000/LConn3 -- bus331/LConn1
  _CN_224209320_275000_CN_75514732_275000/RConn1 -- T_75514732__/LConn1 -- _CN_164675939_275000_CN_75514732_275000/RConn1
  _CN_224209320_275000_CN_75514732_275000/RConn2 -- T_75514732__/LConn2 -- _CN_164675939_275000_CN_75514732_275000/RConn2
  _CN_224209320_275000_CN_75514732_275000/RConn3 -- T_75514732__/LConn3 -- _CN_164675939_275000_CN_75514732_275000/RConn3 -- bus332/LConn1
  _CN_224209320_275000_CN_172364007_275000/RConn1 -- T_172364007__Cherry_Gardens_substation/LConn1 -- _CN_172364007_275000_CN_172867383_275000/LConn1 -- _CN_172364006_275000_CN_172364007_275000/LConn1 -- _CN_172364007_275000_CN_172362099_275000/RConn1
  _CN_224209320_275000_CN_172364007_275000/RConn2 -- T_172364007__Cherry_Gardens_substation/LConn2 -- _CN_172364007_275000_CN_172867383_275000/LConn2 -- _CN_172364006_275000_CN_172364007_275000/LConn2 -- _CN_172364007_275000_CN_172362099_275000/RConn2
  _CN_224209320_275000_CN_172364007_275000/RConn3 -- T_172364007__Cherry_Gardens_substation/LConn3 -- _CN_172364007_275000_CN_172867383_275000/LConn3 -- bus333/LConn1 -- _CN_172364006_275000_CN_172364007_275000/LConn3 -- _CN_172364007_275000_CN_172362099_275000/RConn3
  T_173223683__Abermain_Substation/LConn1 -- _CN_170832455_275000_CN_173223683_275000/RConn1
  T_173223683__Abermain_Substation/LConn2 -- _CN_170832455_275000_CN_173223683_275000/RConn2
  _CN_170832455_275000_CN_173223683_275000/RConn3 -- T_173223683__Abermain_Substation/LConn3 -- bus334/LConn1
  _CN_170058930_275000_CN_164775125_275000/LConn1 -- T_170058930__/LConn1 -- _CN_170058930_275000_CN_120511705_275000/LConn1 -- _CN_170058930_275000_CN_172362099_275000/RConn1 -- _CN_170058930_275000_CN_170036971_275000/LConn1
  _CN_170058930_275000_CN_164775125_275000/LConn2 -- T_170058930__/LConn2 -- _CN_170058930_275000_CN_120511705_275000/LConn2 -- _CN_170058930_275000_CN_172362099_275000/RConn2 -- _CN_170058930_275000_CN_170036971_275000/LConn2
  _CN_170058930_275000_CN_164775125_275000/LConn3 -- T_170058930__/LConn3 -- _CN_170058930_275000_CN_120511705_275000/LConn3 -- _CN_170058930_275000_CN_172362099_275000/RConn3 -- _CN_170058930_275000_CN_170036971_275000/LConn3 -- bus335/LConn1
  T_164775125__/LConn1 -- _CN_170058930_275000_CN_164775125_275000/RConn1
  T_164775125__/LConn2 -- _CN_170058930_275000_CN_164775125_275000/RConn2
  _CN_170058930_275000_CN_164775125_275000/RConn3 -- T_164775125__/LConn3 -- bus336/LConn1
  T_120511705__/LConn1 -- _CN_170058930_275000_CN_120511705_275000/RConn1
  T_120511705__/LConn2 -- _CN_170058930_275000_CN_120511705_275000/RConn2
  _CN_170058930_275000_CN_120511705_275000/RConn3 -- T_120511705__/LConn3 -- bus337/LConn1
  T_170036971__/LConn1 -- _CN_170058930_275000_CN_170036971_275000/RConn1
  T_170036971__/LConn2 -- _CN_170058930_275000_CN_170036971_275000/RConn2
  _CN_170058930_275000_CN_170036971_275000/RConn3 -- T_170036971__/LConn3 -- bus338/LConn1
  _CN_172714955_275000_CN_172714953_275000/RConn1 -- T_172714955__/LConn1 -- _CN_172714955_275000_CN_83656868_275000/LConn1
  _CN_172714955_275000_CN_172714953_275000/RConn2 -- T_172714955__/LConn2 -- _CN_172714955_275000_CN_83656868_275000/LConn2
  _CN_172714955_275000_CN_172714953_275000/RConn3 -- T_172714955__/LConn3 -- _CN_172714955_275000_CN_83656868_275000/LConn3 -- bus339/LConn1
  G_83656868_Pelican_Point_Power_Station/RConn1 -- _CN_172714955_275000_CN_83656868_275000/RConn1
  G_83656868_Pelican_Point_Power_Station/RConn2 -- _CN_172714955_275000_CN_83656868_275000/RConn2
  _CN_172714955_275000_CN_83656868_275000/RConn3 -- G_83656868_Pelican_Point_Power_Station/RConn3 -- bus340/LConn1
  T_165154628__/LConn1 -- _CN_165154628_275000_CN_164764363_275000/LConn1
  T_165154628__/LConn2 -- _CN_165154628_275000_CN_164764363_275000/LConn2
  _CN_165154628_275000_CN_164764363_275000/LConn3 -- T_165154628__/LConn3 -- bus341/LConn1
  T_164764363__/LConn1 -- _CN_165154628_275000_CN_164764363_275000/RConn1
  T_164764363__/LConn2 -- _CN_165154628_275000_CN_164764363_275000/RConn2
  _CN_165154628_275000_CN_164764363_275000/RConn3 -- T_164764363__/LConn3 -- bus342/LConn1
  _CN_196583889_275000_CN_173700961_275000/LConn1 -- T_196583889_275000_275_kV_Chalumbin/LConn1 -- _CN_196583889_275000_CN_171189090_275000/LConn1
  _CN_196583889_275000_CN_173700961_275000/LConn2 -- T_196583889_275000_275_kV_Chalumbin/LConn2 -- _CN_196583889_275000_CN_171189090_275000/LConn2
  _CN_196583889_275000_CN_173700961_275000/LConn3 -- T_196583889_275000_275_kV_Chalumbin/LConn3 -- _CN_196583889_275000_CN_171189090_275000/LConn3 -- bus343/LConn1
  _CN_196583889_275000_CN_173700961_275000/RConn1 -- T_173700961__/LConn1 -- _CN_173700961_275000_CN_189021414_275000/RConn1
  _CN_196583889_275000_CN_173700961_275000/RConn2 -- T_173700961__/LConn2 -- _CN_173700961_275000_CN_189021414_275000/RConn2
  _CN_196583889_275000_CN_173700961_275000/RConn3 -- T_173700961__/LConn3 -- _CN_173700961_275000_CN_189021414_275000/RConn3 -- bus344/LConn1
  T_171189090_275000_275_kV_Ross/LConn1 -- _CN_196583889_275000_CN_171189090_275000/RConn1
  T_171189090_275000_275_kV_Ross/LConn2 -- _CN_196583889_275000_CN_171189090_275000/RConn2
  _CN_196583889_275000_CN_171189090_275000/RConn3 -- T_171189090_275000_275_kV_Ross/LConn3 -- bus345/LConn1
  T_121646942__/LConn1 -- _CN_171486427_275000_CN_121646942_275000/RConn1
  T_121646942__/LConn2 -- _CN_171486427_275000_CN_121646942_275000/RConn2
  _CN_171486427_275000_CN_121646942_275000/RConn3 -- T_121646942__/LConn3 -- bus346/LConn1
  _CN_172364006_275000_CN_172362099_275000/RConn1 -- T_172364006__Electranet_Magill_Substation/LConn1 -- _CN_172364006_275000_CN_172867383_275000/LConn1 -- _CN_172364006_275000_CN_172364007_275000/RConn1
  _CN_172364006_275000_CN_172362099_275000/RConn2 -- T_172364006__Electranet_Magill_Substation/LConn2 -- _CN_172364006_275000_CN_172867383_275000/LConn2 -- _CN_172364006_275000_CN_172364007_275000/RConn2
  _CN_172364006_275000_CN_172362099_275000/RConn3 -- T_172364006__Electranet_Magill_Substation/LConn3 -- _CN_172364006_275000_CN_172867383_275000/LConn3 -- _CN_172364006_275000_CN_172364007_275000/RConn3 -- bus347/LConn1
  _CN_172364006_275000_CN_172867383_275000/RConn1 -- T_172867383__/LConn1 -- _CN_172364007_275000_CN_172867383_275000/RConn1
  _CN_172364006_275000_CN_172867383_275000/RConn2 -- T_172867383__/LConn2 -- _CN_172364007_275000_CN_172867383_275000/RConn2
  _CN_172364006_275000_CN_172867383_275000/RConn3 -- T_172867383__/LConn3 -- _CN_172364007_275000_CN_172867383_275000/RConn3 -- bus348/LConn1
  T_169406848__Wellington_substation/LConn1 -- _CN_169406848_330000_CN_169302216_330000/LConn1
  T_169406848__Wellington_substation/LConn2 -- _CN_169406848_330000_CN_169302216_330000/LConn2
  _CN_169406848_330000_CN_169302216_330000/LConn3 -- T_169406848__Wellington_substation/LConn3 -- bus349/LConn1
  _CN_169406848_330000_CN_169302216_330000/RConn1 -- T_169302216__/RConn1 -- L_169302216/LConn1
  _CN_169406848_330000_CN_169302216_330000/RConn2 -- T_169302216__/RConn2 -- L_169302216/LConn2
  _CN_169406848_330000_CN_169302216_330000/RConn3 -- T_169302216__/RConn3 -- L_169302216/LConn3 -- bus350/LConn1
  _CN_99848705_330000_CN_160201298_330000/LConn1 -- T_99848705_330000_Tamworth_330_132_subtransmission_substation/LConn1 -- _CN_99848705_330000_CN_204894935_330000/LConn1
  _CN_99848705_330000_CN_160201298_330000/LConn2 -- T_99848705_330000_Tamworth_330_132_subtransmission_substation/LConn2 -- _CN_99848705_330000_CN_204894935_330000/LConn2
  _CN_99848705_330000_CN_160201298_330000/LConn3 -- T_99848705_330000_Tamworth_330_132_subtransmission_substation/LConn3 -- _CN_99848705_330000_CN_204894935_330000/LConn3 -- bus351/LConn1
  _CN_99848705_330000_CN_160201298_330000/RConn1 -- T_160201298__Armidale_Substation/LConn1 -- _CN_171853256_330000_CN_160201298_330000/LConn1 -- _CN_172887491_330000_CN_160201298_330000/LConn1
  _CN_99848705_330000_CN_160201298_330000/RConn2 -- T_160201298__Armidale_Substation/LConn2 -- _CN_171853256_330000_CN_160201298_330000/LConn2 -- _CN_172887491_330000_CN_160201298_330000/LConn2
  _CN_99848705_330000_CN_160201298_330000/RConn3 -- T_160201298__Armidale_Substation/LConn3 -- _CN_171853256_330000_CN_160201298_330000/LConn3 -- _CN_172887491_330000_CN_160201298_330000/LConn3 -- bus352/LConn1
  T_204894935__/LConn1 -- _CN_99848705_330000_CN_204894935_330000/RConn1
  T_204894935__/LConn2 -- _CN_99848705_330000_CN_204894935_330000/RConn2
  _CN_99848705_330000_CN_204894935_330000/RConn3 -- T_204894935__/LConn3 -- bus353/LConn1
  _CN_179923658_330000_CN_45237469_330000/LConn1 -- T_179923658__/LConn1 -- _CN_179923658_330000_CN_376493893_330000/LConn1 -- _CN_179923658_330000_CN_24024039_330000/LConn1
  _CN_179923658_330000_CN_45237469_330000/LConn2 -- T_179923658__/LConn2 -- _CN_179923658_330000_CN_376493893_330000/LConn2 -- _CN_179923658_330000_CN_24024039_330000/LConn2
  _CN_179923658_330000_CN_45237469_330000/LConn3 -- T_179923658__/LConn3 -- _CN_179923658_330000_CN_376493893_330000/LConn3 -- _CN_179923658_330000_CN_24024039_330000/LConn3 -- bus354/LConn1
  _CN_179923658_330000_CN_45237469_330000/RConn1 -- T_45237469__Sydney_West_Bulk_Supply_Point/LConn1 -- _CN_376493893_330000_CN_45237469_330000/LConn1 -- _CN_168227360_330000_CN_45237469_330000/LConn1 -- _CN_45237469_330000_CN_203043714_330000/LConn1 -- _CN_45237469_330000_CN_167694317_330000/LConn1
  _CN_179923658_330000_CN_45237469_330000/RConn2 -- T_45237469__Sydney_West_Bulk_Supply_Point/LConn2 -- _CN_376493893_330000_CN_45237469_330000/LConn2 -- _CN_168227360_330000_CN_45237469_330000/LConn2 -- _CN_45237469_330000_CN_203043714_330000/LConn2 -- _CN_45237469_330000_CN_167694317_330000/LConn2
  _CN_179923658_330000_CN_45237469_330000/RConn3 -- T_45237469__Sydney_West_Bulk_Supply_Point/LConn3 -- _CN_376493893_330000_CN_45237469_330000/LConn3 -- _CN_168227360_330000_CN_45237469_330000/LConn3 -- _CN_45237469_330000_CN_203043714_330000/LConn3 -- _CN_45237469_330000_CN_167694317_330000/LConn3 -- bus355/LConn1
  _CN_179923658_330000_CN_376493893_330000/RConn1 -- T_376493893__Vales_Point_Substation/LConn1 -- _CN_376493893_330000_CN_24024039_330000/LConn1 -- _CN_376493893_330000_CN_45237469_330000/RConn1 -- _CN_376493893_330000_CN_24038114_330000/LConn1 -- _CN_376493893_330000_CN_24028364_330000/LConn1
  _CN_179923658_330000_CN_376493893_330000/RConn2 -- T_376493893__Vales_Point_Substation/LConn2 -- _CN_376493893_330000_CN_24024039_330000/LConn2 -- _CN_376493893_330000_CN_45237469_330000/RConn2 -- _CN_376493893_330000_CN_24038114_330000/LConn2 -- _CN_376493893_330000_CN_24028364_330000/LConn2
  _CN_179923658_330000_CN_376493893_330000/RConn3 -- T_376493893__Vales_Point_Substation/LConn3 -- _CN_376493893_330000_CN_24024039_330000/LConn3 -- _CN_376493893_330000_CN_45237469_330000/RConn3 -- _CN_376493893_330000_CN_24038114_330000/LConn3 -- _CN_376493893_330000_CN_24028364_330000/LConn3 -- bus356/LConn1
  _CN_179923658_330000_CN_24024039_330000/RConn1 -- T_24024039__/LConn1 -- _CN_376493893_330000_CN_24024039_330000/RConn1
  _CN_179923658_330000_CN_24024039_330000/RConn2 -- T_24024039__/LConn2 -- _CN_376493893_330000_CN_24024039_330000/RConn2
  _CN_179923658_330000_CN_24024039_330000/RConn3 -- T_24024039__/LConn3 -- _CN_376493893_330000_CN_24024039_330000/RConn3 -- bus357/LConn1
  _CN_87853100_330000_CN_194289858_330000/LConn1 -- T_87853100__/LConn1 -- _CN_87853100_330000_CN_223957157_330000/LConn1
  _CN_87853100_330000_CN_194289858_330000/LConn2 -- T_87853100__/LConn2 -- _CN_87853100_330000_CN_223957157_330000/LConn2
  _CN_87853100_330000_CN_194289858_330000/LConn3 -- T_87853100__/LConn3 -- _CN_87853100_330000_CN_223957157_330000/LConn3 -- bus358/LConn1
  T_194289858__Muja_Switchyard/LConn1 -- _CN_87853100_330000_CN_194289858_330000/RConn1
  T_194289858__Muja_Switchyard/LConn2 -- _CN_87853100_330000_CN_194289858_330000/RConn2
  _CN_87853100_330000_CN_194289858_330000/RConn3 -- T_194289858__Muja_Switchyard/LConn3 -- bus359/LConn1
  T_223957157__/LConn1 -- _CN_87853100_330000_CN_223957157_330000/RConn1
  T_223957157__/LConn2 -- _CN_87853100_330000_CN_223957157_330000/RConn2
  _CN_87853100_330000_CN_223957157_330000/RConn3 -- T_223957157__/LConn3 -- bus360/LConn1
  T_224223244__/LConn1 -- _CN_224223244_330000_CN_44187488_330000/LConn1
  T_224223244__/LConn2 -- _CN_224223244_330000_CN_44187488_330000/LConn2
  _CN_224223244_330000_CN_44187488_330000/LConn3 -- T_224223244__/LConn3 -- bus361/LConn1
  T_44187488__/LConn1 -- _CN_224223244_330000_CN_44187488_330000/RConn1
  T_44187488__/LConn2 -- _CN_224223244_330000_CN_44187488_330000/RConn2
  _CN_224223244_330000_CN_44187488_330000/RConn3 -- T_44187488__/LConn3 -- bus362/LConn1
  T_170842253__Braemar/LConn1 -- _CN_170842253_330000_CN_172887193_330000/LConn1
  T_170842253__Braemar/LConn2 -- _CN_170842253_330000_CN_172887193_330000/LConn2
  _CN_170842253_330000_CN_172887193_330000/LConn3 -- T_170842253__Braemar/LConn3 -- bus363/LConn1
  _CN_170842253_330000_CN_172887193_330000/RConn1 -- T_172887193__Bulli_Creek_substation/LConn1 -- _CN_172887193_330000_CN_170833885_330000/LConn1 -- _CN_172887193_330000_CN_172887491_330000/LConn1
  _CN_170842253_330000_CN_172887193_330000/RConn2 -- T_172887193__Bulli_Creek_substation/LConn2 -- _CN_172887193_330000_CN_170833885_330000/LConn2 -- _CN_172887193_330000_CN_172887491_330000/LConn2
  _CN_170842253_330000_CN_172887193_330000/RConn3 -- T_172887193__Bulli_Creek_substation/LConn3 -- _CN_172887193_330000_CN_170833885_330000/LConn3 -- bus364/LConn1 -- _CN_172887193_330000_CN_172887491_330000/LConn3
  _CN_119871505_330000_CN_160295596_330000/LConn1 -- T_119871505__/LConn1 -- _CN_119871505_330000_CN_160191425_330000/LConn1 -- _CN_119871505_330000_CN_168227360_330000/LConn1
  _CN_119871505_330000_CN_160295596_330000/LConn2 -- T_119871505__/LConn2 -- _CN_119871505_330000_CN_160191425_330000/LConn2 -- _CN_119871505_330000_CN_168227360_330000/LConn2
  _CN_119871505_330000_CN_160295596_330000/LConn3 -- T_119871505__/LConn3 -- _CN_119871505_330000_CN_160191425_330000/LConn3 -- _CN_119871505_330000_CN_168227360_330000/LConn3 -- bus365/LConn1
  _CN_119871505_330000_CN_160295596_330000/RConn1 -- T_160295596_330000;132000_Marulan_Transmission_Substation/LConn1 -- _CN_160295596_330000_CN_172620016_330000/LConn1 -- _CN_160295596_330000_CN_172739944_330000/LConn1
  _CN_119871505_330000_CN_160295596_330000/RConn2 -- T_160295596_330000;132000_Marulan_Transmission_Substation/LConn2 -- _CN_160295596_330000_CN_172620016_330000/LConn2 -- _CN_160295596_330000_CN_172739944_330000/LConn2
  _CN_119871505_330000_CN_160295596_330000/RConn3 -- T_160295596_330000;132000_Marulan_Transmission_Substation/LConn3 -- _CN_160295596_330000_CN_172620016_330000/LConn3 -- _CN_160295596_330000_CN_172739944_330000/LConn3 -- bus366/LConn1
  _CN_119871505_330000_CN_160191425_330000/RConn1 -- T_160191425__/LConn1 -- _CN_160191425_330000_CN_164280399_330000/LConn1
  _CN_119871505_330000_CN_160191425_330000/RConn2 -- T_160191425__/LConn2 -- _CN_160191425_330000_CN_164280399_330000/LConn2
  _CN_119871505_330000_CN_160191425_330000/RConn3 -- T_160191425__/LConn3 -- _CN_160191425_330000_CN_164280399_330000/LConn3 -- bus367/LConn1
  _CN_119871505_330000_CN_168227360_330000/RConn1 -- T_168227360__/LConn1 -- _CN_168227360_330000_CN_45237469_330000/RConn1 -- _CN_168227360_330000_CN_168227361_330000/LConn1
  _CN_119871505_330000_CN_168227360_330000/RConn2 -- T_168227360__/LConn2 -- _CN_168227360_330000_CN_45237469_330000/RConn2 -- _CN_168227360_330000_CN_168227361_330000/LConn2
  _CN_119871505_330000_CN_168227360_330000/RConn3 -- T_168227360__/LConn3 -- _CN_168227360_330000_CN_45237469_330000/RConn3 -- bus368/LConn1 -- _CN_168227360_330000_CN_168227361_330000/LConn3
  T_24038114__/LConn1 -- _CN_376493893_330000_CN_24038114_330000/RConn1
  T_24038114__/LConn2 -- _CN_376493893_330000_CN_24038114_330000/RConn2
  _CN_376493893_330000_CN_24038114_330000/RConn3 -- T_24038114__/LConn3 -- bus369/LConn1
  T_24028364__Newcastle_substation/LConn1 -- _CN_376493893_330000_CN_24028364_330000/RConn1
  T_24028364__Newcastle_substation/LConn2 -- _CN_376493893_330000_CN_24028364_330000/RConn2
  _CN_376493893_330000_CN_24028364_330000/RConn3 -- T_24028364__Newcastle_substation/LConn3 -- bus370/LConn1
  _CN_172887193_330000_CN_172887491_330000/RConn1 -- T_172887491_330000_Dumaresq_switching_station/LConn1 -- _CN_172887491_330000_CN_160201298_330000/RConn1
  _CN_172887193_330000_CN_172887491_330000/RConn2 -- T_172887491_330000_Dumaresq_switching_station/LConn2 -- _CN_172887491_330000_CN_160201298_330000/RConn2
  _CN_172887193_330000_CN_172887491_330000/RConn3 -- T_172887491_330000_Dumaresq_switching_station/LConn3 -- _CN_172887491_330000_CN_160201298_330000/RConn3 -- bus371/LConn1
  _CN_172887193_330000_CN_170833885_330000/RConn1 -- T_170833885__/LConn1 -- _CN_170833885_330000_CN_186721091_330000/LConn1
  _CN_172887193_330000_CN_170833885_330000/RConn2 -- T_170833885__/LConn2 -- _CN_170833885_330000_CN_186721091_330000/LConn2
  _CN_172887193_330000_CN_170833885_330000/RConn3 -- T_170833885__/LConn3 -- _CN_170833885_330000_CN_186721091_330000/LConn3 -- bus372/LConn1
  _CN_168227360_330000_CN_168227361_330000/RConn1 -- T_168227361__/RConn1 -- L_168227361/LConn1
  _CN_168227360_330000_CN_168227361_330000/RConn2 -- T_168227361__/RConn2 -- L_168227361/LConn2
  _CN_168227360_330000_CN_168227361_330000/RConn3 -- T_168227361__/RConn3 -- L_168227361/LConn3 -- bus373/LConn1
  _CN_173873963_330000_CN_175920440_330000/LConn1 -- T_173873963__Kemps_Creek/LConn1 -- _CN_173873963_330000_CN_203043714_330000/LConn1 -- _CN_173873963_330000_CN_172739944_330000/LConn1
  _CN_173873963_330000_CN_175920440_330000/LConn2 -- T_173873963__Kemps_Creek/LConn2 -- _CN_173873963_330000_CN_203043714_330000/LConn2 -- _CN_173873963_330000_CN_172739944_330000/LConn2
  _CN_173873963_330000_CN_175920440_330000/LConn3 -- T_173873963__Kemps_Creek/LConn3 -- _CN_173873963_330000_CN_203043714_330000/LConn3 -- _CN_173873963_330000_CN_172739944_330000/LConn3 -- bus374/LConn1
  _CN_173873963_330000_CN_175920440_330000/RConn1 -- T_175920440__Sydney_South/LConn1 -- _CN_175920440_330000_CN_172620016_330000/LConn1
  _CN_173873963_330000_CN_175920440_330000/RConn2 -- T_175920440__Sydney_South/LConn2 -- _CN_175920440_330000_CN_172620016_330000/LConn2
  _CN_173873963_330000_CN_175920440_330000/RConn3 -- T_175920440__Sydney_South/LConn3 -- _CN_175920440_330000_CN_172620016_330000/LConn3 -- bus375/LConn1
  _CN_173873963_330000_CN_203043714_330000/RConn1 -- T_203043714__/LConn1 -- _CN_45237469_330000_CN_203043714_330000/RConn1
  _CN_173873963_330000_CN_203043714_330000/RConn2 -- T_203043714__/LConn2 -- _CN_45237469_330000_CN_203043714_330000/RConn2
  _CN_173873963_330000_CN_203043714_330000/RConn3 -- T_203043714__/LConn3 -- _CN_45237469_330000_CN_203043714_330000/RConn3 -- bus376/LConn1
  _CN_173873963_330000_CN_172739944_330000/RConn1 -- T_172739944__Avon_Transmission_Substation/LConn1 -- _CN_160295596_330000_CN_172739944_330000/RConn1 -- _CN_172739944_330000_CN_172620016_330000/LConn1
  _CN_173873963_330000_CN_172739944_330000/RConn2 -- T_172739944__Avon_Transmission_Substation/LConn2 -- _CN_160295596_330000_CN_172739944_330000/RConn2 -- _CN_172739944_330000_CN_172620016_330000/LConn2
  _CN_173873963_330000_CN_172739944_330000/RConn3 -- T_172739944__Avon_Transmission_Substation/LConn3 -- _CN_160295596_330000_CN_172739944_330000/RConn3 -- _CN_172739944_330000_CN_172620016_330000/LConn3 -- bus377/LConn1
  _CN_160295596_330000_CN_172620016_330000/RConn1 -- T_172620016_330000;132000_Dapto_Transmission_Substation/LConn1 -- _CN_175920440_330000_CN_172620016_330000/RConn1 -- _CN_172739944_330000_CN_172620016_330000/RConn1
  _CN_160295596_330000_CN_172620016_330000/RConn2 -- T_172620016_330000;132000_Dapto_Transmission_Substation/LConn2 -- _CN_175920440_330000_CN_172620016_330000/RConn2 -- _CN_172739944_330000_CN_172620016_330000/RConn2
  _CN_160295596_330000_CN_172620016_330000/RConn3 -- T_172620016_330000;132000_Dapto_Transmission_Substation/LConn3 -- _CN_175920440_330000_CN_172620016_330000/RConn3 -- _CN_172739944_330000_CN_172620016_330000/RConn3 -- bus378/LConn1
  G_186721091_Millmerran_Power_Station/RConn1 -- _CN_170833885_330000_CN_186721091_330000/RConn1
  G_186721091_Millmerran_Power_Station/RConn2 -- _CN_170833885_330000_CN_186721091_330000/RConn2
  _CN_170833885_330000_CN_186721091_330000/RConn3 -- G_186721091_Millmerran_Power_Station/RConn3 -- bus379/LConn1
  _CN_171853256_330000_CN_160201298_330000/RConn1 -- T_171853256__Coffs_Harbour_subtransmission_station/LConn1 -- _CN_171853256_330000_CN_171581408_330000/LConn1
  _CN_171853256_330000_CN_160201298_330000/RConn2 -- T_171853256__Coffs_Harbour_subtransmission_station/LConn2 -- _CN_171853256_330000_CN_171581408_330000/LConn2
  _CN_171853256_330000_CN_160201298_330000/RConn3 -- T_171853256__Coffs_Harbour_subtransmission_station/LConn3 -- _CN_171853256_330000_CN_171581408_330000/LConn3 -- bus380/LConn1
  T_171581408__Lismore_330_132_subtransmission_station/LConn1 -- _CN_171853256_330000_CN_171581408_330000/RConn1
  T_171581408__Lismore_330_132_subtransmission_station/LConn2 -- _CN_171853256_330000_CN_171581408_330000/RConn2
  _CN_171853256_330000_CN_171581408_330000/RConn3 -- T_171581408__Lismore_330_132_subtransmission_station/LConn3 -- bus381/LConn1
  _CN_173102134_330000_CN_179898706_330000/LConn1 -- T_173102134__/LConn1 -- _CN_173102134_330000_CN_172231145_330000/LConn1
  _CN_173102134_330000_CN_179898706_330000/LConn2 -- T_173102134__/LConn2 -- _CN_173102134_330000_CN_172231145_330000/LConn2
  _CN_173102134_330000_CN_179898706_330000/LConn3 -- T_173102134__/LConn3 -- _CN_173102134_330000_CN_172231145_330000/LConn3 -- bus382/LConn1
  T_179898706__/LConn1 -- _CN_173102134_330000_CN_179898706_330000/RConn1
  T_179898706__/LConn2 -- _CN_173102134_330000_CN_179898706_330000/RConn2
  _CN_173102134_330000_CN_179898706_330000/RConn3 -- T_179898706__/LConn3 -- bus383/LConn1
  _CN_173102134_330000_CN_172231145_330000/RConn1 -- T_172231145__/LConn1 -- _CN_169416665_330000_CN_172231145_330000/LConn1
  _CN_173102134_330000_CN_172231145_330000/RConn2 -- T_172231145__/LConn2 -- _CN_169416665_330000_CN_172231145_330000/LConn2
  _CN_173102134_330000_CN_172231145_330000/RConn3 -- T_172231145__/LConn3 -- _CN_169416665_330000_CN_172231145_330000/LConn3 -- bus384/LConn1
  T_172609354__/LConn1 -- _CN_172609354_330000_CN_170294651_330000/LConn1
  T_172609354__/LConn2 -- _CN_172609354_330000_CN_170294651_330000/LConn2
  _CN_172609354_330000_CN_170294651_330000/LConn3 -- T_172609354__/LConn3 -- bus385/LConn1
  G_170294651_/RConn1 -- _CN_172609354_330000_CN_170294651_330000/RConn1
  G_170294651_/RConn2 -- _CN_172609354_330000_CN_170294651_330000/RConn2
  _CN_172609354_330000_CN_170294651_330000/RConn3 -- G_170294651_/RConn3 -- bus386/LConn1
  T_164280399__/LConn1 -- _CN_160191425_330000_CN_164280399_330000/RConn1
  T_164280399__/LConn2 -- _CN_160191425_330000_CN_164280399_330000/RConn2
  _CN_160191425_330000_CN_164280399_330000/RConn3 -- T_164280399__/LConn3 -- bus387/LConn1
  T_23717060__/LConn1 -- _CN_23717060_330000_CN_286063160_330000/LConn1
  T_23717060__/LConn2 -- _CN_23717060_330000_CN_286063160_330000/LConn2
  _CN_23717060_330000_CN_286063160_330000/LConn3 -- T_23717060__/LConn3 -- bus388/LConn1
  T_286063160__/LConn1 -- _CN_23717060_330000_CN_286063160_330000/RConn1
  T_286063160__/LConn2 -- _CN_23717060_330000_CN_286063160_330000/RConn2
  _CN_23717060_330000_CN_286063160_330000/RConn3 -- T_286063160__/LConn3 -- bus389/LConn1
  T_223943114__/LConn1 -- _CN_223943114_330000_CN_77998934_330000/LConn1
  T_223943114__/LConn2 -- _CN_223943114_330000_CN_77998934_330000/LConn2
  _CN_223943114_330000_CN_77998934_330000/LConn3 -- T_223943114__/LConn3 -- bus390/LConn1
  T_77998934__/LConn1 -- _CN_223943114_330000_CN_77998934_330000/RConn1
  T_77998934__/LConn2 -- _CN_223943114_330000_CN_77998934_330000/RConn2
  _CN_223943114_330000_CN_77998934_330000/RConn3 -- T_77998934__/LConn3 -- bus391/LConn1
  T_45553233__/LConn1 -- _CN_45553233_330000_CN_37106533_330000/LConn1
  T_45553233__/LConn2 -- _CN_45553233_330000_CN_37106533_330000/LConn2
  _CN_45553233_330000_CN_37106533_330000/LConn3 -- T_45553233__/LConn3 -- bus392/LConn1
  T_37106533__/LConn1 -- _CN_45553233_330000_CN_37106533_330000/RConn1
  T_37106533__/LConn2 -- _CN_45553233_330000_CN_37106533_330000/RConn2
  _CN_45553233_330000_CN_37106533_330000/RConn3 -- T_37106533__/LConn3 -- bus393/LConn1
  T_169416665__/LConn1 -- _CN_169416665_330000_CN_172231145_330000/RConn1
  T_169416665__/LConn2 -- _CN_169416665_330000_CN_172231145_330000/RConn2
  _CN_169416665_330000_CN_172231145_330000/RConn3 -- T_169416665__/LConn3 -- bus394/LConn1
  T_167694317__/LConn1 -- _CN_45237469_330000_CN_167694317_330000/RConn1
  T_167694317__/LConn2 -- _CN_45237469_330000_CN_167694317_330000/RConn2
  _CN_45237469_330000_CN_167694317_330000/RConn3 -- T_167694317__/LConn3 -- bus395/LConn1
  T_312550977__AusNet_Tarrone_Terminal_Station/LConn1 -- _CN_312550977_500000_CN_234560801_500000/LConn1
  T_312550977__AusNet_Tarrone_Terminal_Station/LConn2 -- _CN_312550977_500000_CN_234560801_500000/LConn2
  _CN_312550977_500000_CN_234560801_500000/LConn3 -- T_312550977__AusNet_Tarrone_Terminal_Station/LConn3 -- bus396/LConn1
  G_234560801_Origin_Energy_Mortlake_Power_Station/RConn1 -- _CN_312550977_500000_CN_234560801_500000/RConn1
  G_234560801_Origin_Energy_Mortlake_Power_Station/RConn2 -- _CN_312550977_500000_CN_234560801_500000/RConn2
  _CN_312550977_500000_CN_234560801_500000/RConn3 -- G_234560801_Origin_Energy_Mortlake_Power_Station/RConn3 -- bus397/LConn1
  T_24054804__SP_AusNet_Rowville_Terminal_Station/LConn1 -- _CN_24054804_500000_CN_48955336_500000/LConn1
  T_24054804__SP_AusNet_Rowville_Terminal_Station/LConn2 -- _CN_24054804_500000_CN_48955336_500000/LConn2
  _CN_24054804_500000_CN_48955336_500000/LConn3 -- T_24054804__SP_AusNet_Rowville_Terminal_Station/LConn3 -- bus398/LConn1
  _CN_24054804_500000_CN_48955336_500000/RConn1 -- T_48955336__SP_AusNet_Cranbourne_Terminal_Station/LConn1 -- _CN_146581916_500000_CN_48955336_500000/LConn1
  _CN_24054804_500000_CN_48955336_500000/RConn2 -- T_48955336__SP_AusNet_Cranbourne_Terminal_Station/LConn2 -- _CN_146581916_500000_CN_48955336_500000/LConn2
  _CN_24054804_500000_CN_48955336_500000/RConn3 -- T_48955336__SP_AusNet_Cranbourne_Terminal_Station/LConn3 -- _CN_146581916_500000_CN_48955336_500000/LConn3 -- bus399/LConn1
  _CN_146581911_500000_CN_146581916_500000/LConn1 -- T_146581911__/LConn1 -- _CN_146581911_500000_CN_146579820_500000/LConn1
  _CN_146581911_500000_CN_146581916_500000/LConn2 -- T_146581911__/LConn2 -- _CN_146581911_500000_CN_146579820_500000/LConn2
  _CN_146581911_500000_CN_146581916_500000/LConn3 -- T_146581911__/LConn3 -- _CN_146581911_500000_CN_146579820_500000/LConn3 -- bus400/LConn1
  _CN_146581911_500000_CN_146581916_500000/RConn1 -- T_146581916_500000_/LConn1 -- _CN_146581916_500000_CN_48955336_500000/RConn1 -- _CN_146581916_500000_CN_23717059_500000/LConn1
  _CN_146581911_500000_CN_146581916_500000/RConn2 -- T_146581916_500000_/LConn2 -- _CN_146581916_500000_CN_48955336_500000/RConn2 -- _CN_146581916_500000_CN_23717059_500000/LConn2
  _CN_146581911_500000_CN_146581916_500000/RConn3 -- T_146581916_500000_/LConn3 -- _CN_146581916_500000_CN_48955336_500000/RConn3 -- _CN_146581916_500000_CN_23717059_500000/LConn3 -- bus401/LConn1
  T_146579820__Loy_Yang_HVDC_Converter/LConn1 -- _CN_146581911_500000_CN_146579820_500000/RConn1
  T_146579820__Loy_Yang_HVDC_Converter/LConn2 -- _CN_146581911_500000_CN_146579820_500000/RConn2
  _CN_146581911_500000_CN_146579820_500000/RConn3 -- T_146579820__Loy_Yang_HVDC_Converter/LConn3 -- bus402/LConn1
  _CN_146581916_500000_CN_23717059_500000/RConn1 -- T_23717059__/LConn1 -- _CN_49455810_500000_CN_23717059_500000/LConn1 -- _CN_23717059_500000_CN_21239912_500000/LConn1
  _CN_146581916_500000_CN_23717059_500000/RConn2 -- T_23717059__/LConn2 -- _CN_49455810_500000_CN_23717059_500000/LConn2 -- _CN_23717059_500000_CN_21239912_500000/LConn2
  _CN_146581916_500000_CN_23717059_500000/RConn3 -- T_23717059__/LConn3 -- _CN_49455810_500000_CN_23717059_500000/LConn3 -- _CN_23717059_500000_CN_21239912_500000/LConn3 -- bus403/LConn1
  T_168227361__/LConn1 -- _CN_168227361_500000_CN_169408193_500000/LConn1
  T_168227361__/LConn2 -- _CN_168227361_500000_CN_169408193_500000/LConn2
  _CN_168227361_500000_CN_169408193_500000/LConn3 -- T_168227361__/LConn3 -- bus404/LConn1
  _CN_168227361_500000_CN_169408193_500000/RConn1 -- T_169408193__/LConn1 -- _CN_169302216_500000_CN_169408193_500000/LConn1
  _CN_168227361_500000_CN_169408193_500000/RConn2 -- T_169408193__/LConn2 -- _CN_169302216_500000_CN_169408193_500000/LConn2
  _CN_168227361_500000_CN_169408193_500000/RConn3 -- T_169408193__/LConn3 -- _CN_169302216_500000_CN_169408193_500000/LConn3 -- bus405/LConn1
  T_23647798__SP_AusNet_Sydenham_Terminal_Station/LConn1 -- _CN_23647798_500000_CN_21239912_500000/LConn1
  T_23647798__SP_AusNet_Sydenham_Terminal_Station/LConn2 -- _CN_23647798_500000_CN_21239912_500000/LConn2
  _CN_23647798_500000_CN_21239912_500000/LConn3 -- T_23647798__SP_AusNet_Sydenham_Terminal_Station/LConn3 -- bus406/LConn1
  _CN_23647798_500000_CN_21239912_500000/RConn1 -- T_21239912__AusNet_Keilor_Terminal_Station/LConn1 -- _CN_23717059_500000_CN_21239912_500000/RConn1
  _CN_23647798_500000_CN_21239912_500000/RConn2 -- T_21239912__AusNet_Keilor_Terminal_Station/LConn2 -- _CN_23717059_500000_CN_21239912_500000/RConn2
  _CN_23647798_500000_CN_21239912_500000/RConn3 -- T_21239912__AusNet_Keilor_Terminal_Station/LConn3 -- _CN_23717059_500000_CN_21239912_500000/RConn3 -- bus407/LConn1
  T_169302216__/LConn1 -- _CN_169302216_500000_CN_169408193_500000/RConn1
  T_169302216__/LConn2 -- _CN_169302216_500000_CN_169408193_500000/RConn2
  _CN_169302216_500000_CN_169408193_500000/RConn3 -- T_169302216__/LConn3 -- bus408/LConn1
  T_49455810__Moorabool_Terminal_Station/LConn1 -- _CN_49455810_500000_CN_23717059_500000/RConn1
  T_49455810__Moorabool_Terminal_Station/LConn2 -- _CN_49455810_500000_CN_23717059_500000/RConn2
  _CN_49455810_500000_CN_23717059_500000/RConn3 -- T_49455810__Moorabool_Terminal_Station/LConn3 -- bus409/LConn1
  T_305092097__/RConn1 -- L_305092097/LConn1
  T_305092097__/RConn2 -- L_305092097/LConn2
  L_305092097/LConn3 -- T_305092097__/RConn3 -- bus410/LConn1
  T_305092094__/RConn1 -- L_305092094/LConn1
  T_305092094__/RConn2 -- L_305092094/LConn2
  L_305092094/LConn3 -- T_305092094__/RConn3 -- bus411/LConn1
  T_303420374__Richlands_Substation/RConn1 -- L_303420374/LConn1
  T_303420374__Richlands_Substation/RConn2 -- L_303420374/LConn2
  L_303420374/LConn3 -- T_303420374__Richlands_Substation/RConn3 -- bus412/LConn1
  T_46146107__Algester_Substation/RConn1 -- L_46146107/LConn1
  T_46146107__Algester_Substation/RConn2 -- L_46146107/LConn2
  L_46146107/LConn3 -- T_46146107__Algester_Substation/RConn3 -- bus413/LConn1
  T_19388439__West_Darra_Substation/RConn1 -- L_19388439/LConn1
  T_19388439__West_Darra_Substation/RConn2 -- L_19388439/LConn2
  L_19388439/LConn3 -- T_19388439__West_Darra_Substation/RConn3 -- bus414/LConn1
  T_303417152__Sumner_Substation/RConn1 -- L_303417152/LConn1
  T_303417152__Sumner_Substation/RConn2 -- L_303417152/LConn2
  L_303417152/LConn3 -- T_303417152__Sumner_Substation/RConn3 -- bus415/LConn1
  T_162321863__/RConn1 -- L_162321863/LConn1
  T_162321863__/RConn2 -- L_162321863/LConn2
  L_162321863/LConn3 -- T_162321863__/RConn3 -- bus416/LConn1
  T_372546567__/RConn1 -- L_372546567/LConn1
  T_372546567__/RConn2 -- L_372546567/LConn2
  L_372546567/LConn3 -- T_372546567__/RConn3 -- bus417/LConn1
  T_23171307__/RConn1 -- L_23171307/LConn1
  T_23171307__/RConn2 -- L_23171307/LConn2
  L_23171307/LConn3 -- T_23171307__/RConn3 -- bus418/LConn1
  T_233929226__/RConn1 -- L_233929226/LConn1
  T_233929226__/RConn2 -- L_233929226/LConn2
  L_233929226/LConn3 -- T_233929226__/RConn3 -- bus419/LConn1
  T_435794582__Tungatinah_Switchyard/RConn1 -- L_435794582/LConn1
  T_435794582__Tungatinah_Switchyard/RConn2 -- L_435794582/LConn2
  L_435794582/LConn3 -- T_435794582__Tungatinah_Switchyard/RConn3 -- bus420/LConn1
  T_23239876__/RConn1 -- L_23239876/LConn1
  T_23239876__/RConn2 -- L_23239876/LConn2
  L_23239876/LConn3 -- T_23239876__/RConn3 -- bus421/LConn1
  T_175926350__/RConn1 -- L_175926350/LConn1
  T_175926350__/RConn2 -- L_175926350/LConn2
  L_175926350/LConn3 -- T_175926350__/RConn3 -- bus422/LConn1
  T_233927398__/RConn1 -- L_233927398/LConn1
  T_233927398__/RConn2 -- L_233927398/LConn2
  L_233927398/LConn3 -- T_233927398__/RConn3 -- bus423/LConn1
  T_233927458__/RConn1 -- L_233927458/LConn1
  T_233927458__/RConn2 -- L_233927458/LConn2
  L_233927458/LConn3 -- T_233927458__/RConn3 -- bus424/LConn1
  T_374644110__/RConn1 -- L_374644110/LConn1
  T_374644110__/RConn2 -- L_374644110/LConn2
  L_374644110/LConn3 -- T_374644110__/RConn3 -- bus425/LConn1
  T_46056595__/RConn1 -- L_46056595/LConn1
  T_46056595__/RConn2 -- L_46056595/LConn2
  L_46056595/LConn3 -- T_46056595__/RConn3 -- bus426/LConn1
  T_171582113__/RConn1 -- L_171582113/LConn1
  T_171582113__/RConn2 -- L_171582113/LConn2
  L_171582113/LConn3 -- T_171582113__/RConn3 -- bus427/LConn1
  T_308160583__Gatton_North_Substation/RConn1 -- L_308160583/LConn1
  T_308160583__Gatton_North_Substation/RConn2 -- L_308160583/LConn2
  L_308160583/LConn3 -- T_308160583__Gatton_North_Substation/RConn3 -- bus428/LConn1
  T_308160585__Postmans_Ridge_Substation/RConn1 -- L_308160585/LConn1
  T_308160585__Postmans_Ridge_Substation/RConn2 -- L_308160585/LConn2
  L_308160585/LConn3 -- T_308160585__Postmans_Ridge_Substation/RConn3 -- bus429/LConn1
  T_66035178__Lockrose_Substation/RConn1 -- L_66035178/LConn1
  T_66035178__Lockrose_Substation/RConn2 -- L_66035178/LConn2
  L_66035178/LConn3 -- T_66035178__Lockrose_Substation/RConn3 -- bus430/LConn1
  T_46305863__Goodna_Substation/RConn1 -- L_46305863/LConn1
  T_46305863__Goodna_Substation/RConn2 -- L_46305863/LConn2
  L_46305863/LConn3 -- T_46305863__Goodna_Substation/RConn3 -- bus431/LConn1
  T_19386719__/RConn1 -- L_19386719/LConn1
  T_19386719__/RConn2 -- L_19386719/LConn2
  L_19386719/LConn3 -- T_19386719__/RConn3 -- bus432/LConn1
  T_26204314__Redbank_Plains_Substation/RConn1 -- L_26204314/LConn1
  T_26204314__Redbank_Plains_Substation/RConn2 -- L_26204314/LConn2
  L_26204314/LConn3 -- T_26204314__Redbank_Plains_Substation/RConn3 -- bus433/LConn1
  T_26161587__Runcorn_Substation/RConn1 -- L_26161587/LConn1
  T_26161587__Runcorn_Substation/RConn2 -- L_26161587/LConn2
  L_26161587/LConn3 -- T_26161587__Runcorn_Substation/RConn3 -- bus434/LConn1
  T_234083162__/RConn1 -- L_234083162/LConn1
  T_234083162__/RConn2 -- L_234083162/LConn2
  L_234083162/LConn3 -- T_234083162__/RConn3 -- bus435/LConn1
  T_234083164__/RConn1 -- L_234083164/LConn1
  T_234083164__/RConn2 -- L_234083164/LConn2
  L_234083164/LConn3 -- T_234083164__/RConn3 -- bus436/LConn1
  T_171575462__/RConn1 -- L_171575462/LConn1
  T_171575462__/RConn2 -- L_171575462/LConn2
  L_171575462/LConn3 -- T_171575462__/RConn3 -- bus437/LConn1
  T_171575468__/RConn1 -- L_171575468/LConn1
  T_171575468__/RConn2 -- L_171575468/LConn2
  L_171575468/LConn3 -- T_171575468__/RConn3 -- bus438/LConn1
  T_174431697__Devonport_Substation/RConn1 -- L_174431697/LConn1
  T_174431697__Devonport_Substation/RConn2 -- L_174431697/LConn2
  L_174431697/LConn3 -- T_174431697__Devonport_Substation/RConn3 -- bus439/LConn1
  T_175174348__/RConn1 -- L_175174348/LConn1
  T_175174348__/RConn2 -- L_175174348/LConn2
  L_175174348/LConn3 -- T_175174348__/RConn3 -- bus440/LConn1
  T_46339655__/RConn1 -- L_46339655/LConn1
  T_46339655__/RConn2 -- L_46339655/LConn2
  L_46339655/LConn3 -- T_46339655__/RConn3 -- bus441/LConn1
  T_258723245__/RConn1 -- L_258723245/LConn1
  T_258723245__/RConn2 -- L_258723245/LConn2
  L_258723245/LConn3 -- T_258723245__/RConn3 -- bus442/LConn1
  T_168385464__/RConn1 -- L_168385464/LConn1
  T_168385464__/RConn2 -- L_168385464/LConn2
  L_168385464/LConn3 -- T_168385464__/RConn3 -- bus443/LConn1
  T_176275951__/RConn1 -- L_176275951/LConn1
  T_176275951__/RConn2 -- L_176275951/LConn2
  L_176275951/LConn3 -- T_176275951__/RConn3 -- bus444/LConn1
  T_173094501__South_Toowoomba/RConn1 -- L_173094501/LConn1
  T_173094501__South_Toowoomba/RConn2 -- L_173094501/LConn2
  L_173094501/LConn3 -- T_173094501__South_Toowoomba/RConn3 -- bus445/LConn1
  T_19388978__Rocklea_Substation/RConn1 -- L_19388978/LConn1
  T_19388978__Rocklea_Substation/RConn2 -- L_19388978/LConn2
  L_19388978/LConn3 -- T_19388978__Rocklea_Substation/RConn3 -- bus446/LConn1
  T_302351763__Archerfield_Substation/RConn1 -- L_302351763/LConn1
  T_302351763__Archerfield_Substation/RConn2 -- L_302351763/LConn2
  L_302351763/LConn3 -- T_302351763__Archerfield_Substation/RConn3 -- bus447/LConn1
  T_175927476__/RConn1 -- L_175927476/LConn1
  T_175927476__/RConn2 -- L_175927476/LConn2
  L_175927476/LConn3 -- T_175927476__/RConn3 -- bus448/LConn1
  T_175926345__New_Norfolk_Substation/RConn1 -- L_175926345/LConn1
  T_175926345__New_Norfolk_Substation/RConn2 -- L_175926345/LConn2
  L_175926345/LConn3 -- T_175926345__New_Norfolk_Substation/RConn3 -- bus449/LConn1
  T_125600603__Robina_Substation/RConn1 -- L_125600603/LConn1
  T_125600603__Robina_Substation/RConn2 -- L_125600603/LConn2
  L_125600603/LConn3 -- T_125600603__Robina_Substation/RConn3 -- bus450/LConn1
  T_30471365__/RConn1 -- L_30471365/LConn1
  T_30471365__/RConn2 -- L_30471365/LConn2
  L_30471365/LConn3 -- T_30471365__/RConn3 -- bus451/LConn1
  T_48853232__/RConn1 -- L_48853232/LConn1
  T_48853232__/RConn2 -- L_48853232/LConn2
  L_48853232/LConn3 -- T_48853232__/RConn3 -- bus452/LConn1
  T_171581686__/RConn1 -- L_171581686/LConn1
  T_171581686__/RConn2 -- L_171581686/LConn2
  L_171581686/LConn3 -- T_171581686__/RConn3 -- bus453/LConn1
  T_307100131__/RConn1 -- L_307100131/LConn1
  T_307100131__/RConn2 -- L_307100131/LConn2
  L_307100131/LConn3 -- T_307100131__/RConn3 -- bus454/LConn1
  T_155682345__Stradbroke_Island_Substation/RConn1 -- L_155682345/LConn1
  T_155682345__Stradbroke_Island_Substation/RConn2 -- L_155682345/LConn2
  L_155682345/LConn3 -- T_155682345__Stradbroke_Island_Substation/RConn3 -- bus455/LConn1
  T_234083565__/RConn1 -- L_234083565/LConn1
  T_234083565__/RConn2 -- L_234083565/LConn2
  L_234083565/LConn3 -- T_234083565__/RConn3 -- bus456/LConn1
  T_234863481__/RConn1 -- L_234863481/LConn1
  T_234863481__/RConn2 -- L_234863481/LConn2
  L_234863481/LConn3 -- T_234863481__/RConn3 -- bus457/LConn1
  T_234176499__/RConn1 -- L_234176499/LConn1
  T_234176499__/RConn2 -- L_234176499/LConn2
  L_234176499/LConn3 -- T_234176499__/RConn3 -- bus458/LConn1
  T_173730623_132000_Tamworth_132_66_subtransmission_substation/RConn1 -- L_173730623/LConn1
  T_173730623_132000_Tamworth_132_66_subtransmission_substation/RConn2 -- L_173730623/LConn2
  L_173730623/LConn3 -- T_173730623_132000_Tamworth_132_66_subtransmission_substation/RConn3 -- bus459/LConn1
  T_366327501_132000_Gunnedah_subtransmission_substation/RConn1 -- L_366327501/LConn1
  T_366327501_132000_Gunnedah_subtransmission_substation/RConn2 -- L_366327501/LConn2
  L_366327501/LConn3 -- T_366327501_132000_Gunnedah_subtransmission_substation/RConn3 -- bus460/LConn1
  T_171582472__/RConn1 -- L_171582472/LConn1
  T_171582472__/RConn2 -- L_171582472/LConn2
  L_171582472/LConn3 -- T_171582472__/RConn3 -- bus461/LConn1
  T_171588475__Chinchilla_Substation/RConn1 -- L_171588475/LConn1
  T_171588475__Chinchilla_Substation/RConn2 -- L_171588475/LConn2
  L_171588475/LConn3 -- T_171588475__Chinchilla_Substation/RConn3 -- bus462/LConn1
  T_194550809__/RConn1 -- L_194550809/LConn1
  T_194550809__/RConn2 -- L_194550809/LConn2
  L_194550809/LConn3 -- T_194550809__/RConn3 -- bus463/LConn1
  T_194550807__/RConn1 -- L_194550807/LConn1
  T_194550807__/RConn2 -- L_194550807/LConn2
  L_194550807/LConn3 -- T_194550807__/RConn3 -- bus464/LConn1
  T_189021048__132_kV_Turkinje/RConn1 -- L_189021048/LConn1
  T_189021048__132_kV_Turkinje/RConn2 -- L_189021048/LConn2
  L_189021048/LConn3 -- T_189021048__132_kV_Turkinje/RConn3 -- bus465/LConn1
  T_173224446_132000_132_kV_Innisfail/RConn1 -- L_173224446/LConn1
  T_173224446_132000_132_kV_Innisfail/RConn2 -- L_173224446/LConn2
  L_173224446/LConn3 -- T_173224446_132000_132_kV_Innisfail/RConn3 -- bus466/LConn1
  T_173224184_132000_132_kV_El_Arish/RConn1 -- L_173224184/LConn1
  T_173224184_132000_132_kV_El_Arish/RConn2 -- L_173224184/LConn2
  L_173224184/LConn3 -- T_173224184_132000_132_kV_El_Arish/RConn3 -- bus467/LConn1
  T_196583888_132000_132_kV_Tully/RConn1 -- L_196583888/LConn1
  T_196583888_132000_132_kV_Tully/RConn2 -- L_196583888/LConn2
  L_196583888/LConn3 -- T_196583888_132000_132_kV_Tully/RConn3 -- bus468/LConn1
  T_196020053_132000_132_kV_Edmonton/RConn1 -- L_196020053/LConn1
  T_196020053_132000_132_kV_Edmonton/RConn2 -- L_196020053/LConn2
  L_196020053/LConn3 -- T_196020053_132000_132_kV_Edmonton/RConn3 -- bus469/LConn1
  T_173396697__/RConn1 -- L_173396697/LConn1
  T_173396697__/RConn2 -- L_173396697/LConn2
  L_173396697/LConn3 -- T_173396697__/RConn3 -- bus470/LConn1
  T_205012494__/RConn1 -- L_205012494/LConn1
  T_205012494__/RConn2 -- L_205012494/LConn2
  L_205012494/LConn3 -- T_205012494__/RConn3 -- bus471/LConn1
  T_205012488__/RConn1 -- L_205012488/LConn1
  T_205012488__/RConn2 -- L_205012488/LConn2
  L_205012488/LConn3 -- T_205012488__/RConn3 -- bus472/LConn1
  T_344076960__/RConn1 -- L_344076960/LConn1
  T_344076960__/RConn2 -- L_344076960/LConn2
  L_344076960/LConn3 -- T_344076960__/RConn3 -- bus473/LConn1
  T_174036841__Cowra_substation/RConn1 -- L_174036841/LConn1
  T_174036841__Cowra_substation/RConn2 -- L_174036841/LConn2
  L_174036841/LConn3 -- T_174036841__Cowra_substation/RConn3 -- bus474/LConn1
  T_214977199__/RConn1 -- L_214977199/LConn1
  T_214977199__/RConn2 -- L_214977199/LConn2
  L_214977199/LConn3 -- T_214977199__/RConn3 -- bus475/LConn1
  T_166192455__/RConn1 -- L_166192455/LConn1
  T_166192455__/RConn2 -- L_166192455/LConn2
  L_166192455/LConn3 -- T_166192455__/RConn3 -- bus476/LConn1
  T_163374878__Bruce_Substation/RConn1 -- L_163374878/LConn1
  T_163374878__Bruce_Substation/RConn2 -- L_163374878/LConn2
  L_163374878/LConn3 -- T_163374878__Bruce_Substation/RConn3 -- bus477/LConn1
  T_192353822_132000;66000;22000_Lakeland_Substation/RConn1 -- L_192353822/LConn1
  T_192353822_132000;66000;22000_Lakeland_Substation/RConn2 -- L_192353822/LConn2
  L_192353822/LConn3 -- T_192353822_132000;66000;22000_Lakeland_Substation/RConn3 -- bus478/LConn1
  T_191779550__/RConn1 -- L_191779550/LConn1
  T_191779550__/RConn2 -- L_191779550/LConn2
  L_191779550/LConn3 -- T_191779550__/RConn3 -- bus479/LConn1
  T_232106017__/RConn1 -- L_232106017/LConn1
  T_232106017__/RConn2 -- L_232106017/LConn2
  L_232106017/LConn3 -- T_232106017__/RConn3 -- bus480/LConn1
  T_232109241__Williamsdale/RConn1 -- L_232109241/LConn1
  T_232109241__Williamsdale/RConn2 -- L_232109241/LConn2
  L_232109241/LConn3 -- T_232109241__Williamsdale/RConn3 -- bus481/LConn1
  T_172230182__/RConn1 -- L_172230182/LConn1
  T_172230182__/RConn2 -- L_172230182/LConn2
  L_172230182/LConn3 -- T_172230182__/RConn3 -- bus482/LConn1
  T_234539007__Glen_Innes_subtransmission_station/RConn1 -- L_234539007/LConn1
  T_234539007__Glen_Innes_subtransmission_station/RConn2 -- L_234539007/LConn2
  L_234539007/LConn3 -- T_234539007__Glen_Innes_subtransmission_station/RConn3 -- bus483/LConn1
  T_340560031__Tenterfield_subtransmission_station/RConn1 -- L_340560031/LConn1
  T_340560031__Tenterfield_subtransmission_station/RConn2 -- L_340560031/LConn2
  L_340560031/LConn3 -- T_340560031__Tenterfield_subtransmission_station/RConn3 -- bus484/LConn1
  T_179921457__Belrose_Substation/RConn1 -- L_179921457/LConn1
  T_179921457__Belrose_Substation/RConn2 -- L_179921457/LConn2
  L_179921457/LConn3 -- T_179921457__Belrose_Substation/RConn3 -- bus485/LConn1
  T_175862605__/RConn1 -- L_175862605/LConn1
  T_175862605__/RConn2 -- L_175862605/LConn2
  L_175862605/LConn3 -- T_175862605__/RConn3 -- bus486/LConn1
  T_45727589__/RConn1 -- L_45727589/LConn1
  T_45727589__/RConn2 -- L_45727589/LConn2
  L_45727589/LConn3 -- T_45727589__/RConn3 -- bus487/LConn1
  T_224223242__/RConn1 -- L_224223242/LConn1
  T_224223242__/RConn2 -- L_224223242/LConn2
  L_224223242/LConn3 -- T_224223242__/RConn3 -- bus488/LConn1
  T_44192327__/RConn1 -- L_44192327/LConn1
  T_44192327__/RConn2 -- L_44192327/LConn2
  L_44192327/LConn3 -- T_44192327__/RConn3 -- bus489/LConn1
  T_164764211__/RConn1 -- L_164764211/LConn1
  T_164764211__/RConn2 -- L_164764211/LConn2
  L_164764211/LConn3 -- T_164764211__/RConn3 -- bus490/LConn1
  T_169687537__Keith_substation/RConn1 -- L_169687537/LConn1
  T_169687537__Keith_substation/RConn2 -- L_169687537/LConn2
  L_169687537/LConn3 -- T_169687537__Keith_substation/RConn3 -- bus491/LConn1
  T_267376693__Bateman's_Bay/RConn1 -- L_267376693/LConn1
  T_267376693__Bateman's_Bay/RConn2 -- L_267376693/LConn2
  L_267376693/LConn3 -- T_267376693__Bateman's_Bay/RConn3 -- bus492/LConn1
  T_267376695__Evans_Lane_Zone_Substation/RConn1 -- L_267376695/LConn1
  T_267376695__Evans_Lane_Zone_Substation/RConn2 -- L_267376695/LConn2
  L_267376695/LConn3 -- T_267376695__Evans_Lane_Zone_Substation/RConn3 -- bus493/LConn1
  T_267376701__/RConn1 -- L_267376701/LConn1
  T_267376701__/RConn2 -- L_267376701/LConn2
  L_267376701/LConn3 -- T_267376701__/RConn3 -- bus494/LConn1
  T_174835009__/RConn1 -- L_174835009/LConn1
  T_174835009__/RConn2 -- L_174835009/LConn2
  L_174835009/LConn3 -- T_174835009__/RConn3 -- bus495/LConn1
  T_174831245__/RConn1 -- L_174831245/LConn1
  T_174831245__/RConn2 -- L_174831245/LConn2
  L_174831245/LConn3 -- T_174831245__/RConn3 -- bus496/LConn1
  T_267376699__Ulladulla_Zone_Substation/RConn1 -- L_267376699/LConn1
  T_267376699__Ulladulla_Zone_Substation/RConn2 -- L_267376699/LConn2
  L_267376699/LConn3 -- T_267376699__Ulladulla_Zone_Substation/RConn3 -- bus497/LConn1
  T_267376698_132000;33000_Shoalhaven_Transmission_Substation/RConn1 -- L_267376698/LConn1
  T_267376698_132000;33000_Shoalhaven_Transmission_Substation/RConn2 -- L_267376698/LConn2
  L_267376698/LConn3 -- T_267376698_132000;33000_Shoalhaven_Transmission_Substation/RConn3 -- bus498/LConn1
  T_174124088__/RConn1 -- L_174124088/LConn1
  T_174124088__/RConn2 -- L_174124088/LConn2
  L_174124088/LConn3 -- T_174124088__/RConn3 -- bus499/LConn1
  T_171746362__/RConn1 -- L_171746362/LConn1
  T_171746362__/RConn2 -- L_171746362/LConn2
  L_171746362/LConn3 -- T_171746362__/RConn3 -- bus500/LConn1
  T_171744984__/RConn1 -- L_171744984/LConn1
  T_171744984__/RConn2 -- L_171744984/LConn2
  L_171744984/LConn3 -- T_171744984__/RConn3 -- bus501/LConn1
  T_366321212_132000_Moree_subtransmission_substation/RConn1 -- L_366321212/LConn1
  T_366321212_132000_Moree_subtransmission_substation/RConn2 -- L_366321212/LConn2
  L_366321212/LConn3 -- T_366321212_132000_Moree_subtransmission_substation/RConn3 -- bus502/LConn1
  T_172891041__Inverell_subtransmission_station/RConn1 -- L_172891041/LConn1
  T_172891041__Inverell_subtransmission_station/RConn2 -- L_172891041/LConn2
  L_172891041/LConn3 -- T_172891041__Inverell_subtransmission_station/RConn3 -- bus503/LConn1
  T_366605305_132000_Narrabri_subtransmission_substation/RConn1 -- L_366605305/LConn1
  T_366605305_132000_Narrabri_subtransmission_substation/RConn2 -- L_366605305/LConn2
  L_366605305/LConn3 -- T_366605305_132000_Narrabri_subtransmission_substation/RConn3 -- bus504/LConn1
  T_47069245__Mount_Lawley_sub_station/RConn1 -- L_47069245/LConn1
  T_47069245__Mount_Lawley_sub_station/RConn2 -- L_47069245/LConn2
  L_47069245/LConn3 -- T_47069245__Mount_Lawley_sub_station/RConn3 -- bus505/LConn1
  T_45402899__/RConn1 -- L_45402899/LConn1
  T_45402899__/RConn2 -- L_45402899/LConn2
  L_45402899/LConn3 -- T_45402899__/RConn3 -- bus506/LConn1
  T_145689826__/RConn1 -- L_145689826/LConn1
  T_145689826__/RConn2 -- L_145689826/LConn2
  L_145689826/LConn3 -- T_145689826__/RConn3 -- bus507/LConn1
  T_171852863__/RConn1 -- L_171852863/LConn1
  T_171852863__/RConn2 -- L_171852863/LConn2
  L_171852863/LConn3 -- T_171852863__/RConn3 -- bus508/LConn1
  T_72231236__/RConn1 -- L_72231236/LConn1
  T_72231236__/RConn2 -- L_72231236/LConn2
  L_72231236/LConn3 -- T_72231236__/RConn3 -- bus509/LConn1
  T_312679496__Macarthur_Wind_Farm_Substation/RConn1 -- L_312679496/LConn1
  T_312679496__Macarthur_Wind_Farm_Substation/RConn2 -- L_312679496/LConn2
  L_312679496/LConn3 -- T_312679496__Macarthur_Wind_Farm_Substation/RConn3 -- bus510/LConn1
  T_312551365__/RConn1 -- L_312551365/LConn1
  T_312551365__/RConn2 -- L_312551365/LConn2
  L_312551365/LConn3 -- T_312551365__/RConn3 -- bus511/LConn1
  T_48579657__/RConn1 -- L_48579657/LConn1
  T_48579657__/RConn2 -- L_48579657/LConn2
  L_48579657/LConn3 -- T_48579657__/RConn3 -- bus512/LConn1
  T_133353043__/RConn1 -- L_133353043/LConn1
  T_133353043__/RConn2 -- L_133353043/LConn2
  L_133353043/LConn3 -- T_133353043__/RConn3 -- bus513/LConn1
  T_47036496__/RConn1 -- L_47036496/LConn1
  T_47036496__/RConn2 -- L_47036496/LConn2
  L_47036496/LConn3 -- T_47036496__/RConn3 -- bus514/LConn1
  T_37106603__/RConn1 -- L_37106603/LConn1
  T_37106603__/RConn2 -- L_37106603/LConn2
  L_37106603/LConn3 -- T_37106603__/RConn3 -- bus515/LConn1
  T_171962240_132000_Koolkhan_subtransmission_substation/RConn1 -- L_171962240/LConn1
  T_171962240_132000_Koolkhan_subtransmission_substation/RConn2 -- L_171962240/LConn2
  L_171962240/LConn3 -- T_171962240_132000_Koolkhan_subtransmission_substation/RConn3 -- bus516/LConn1
  T_44140812__/RConn1 -- L_44140812/LConn1
  T_44140812__/RConn2 -- L_44140812/LConn2
  L_44140812/LConn3 -- T_44140812__/RConn3 -- bus517/LConn1
  T_214229754__/RConn1 -- L_214229754/LConn1
  T_214229754__/RConn2 -- L_214229754/LConn2
  L_214229754/LConn3 -- T_214229754__/RConn3 -- bus518/LConn1
  T_231510030__/RConn1 -- L_231510030/LConn1
  T_231510030__/RConn2 -- L_231510030/LConn2
  L_231510030/LConn3 -- T_231510030__/RConn3 -- bus519/LConn1
  T_170066302__/RConn1 -- L_170066302/LConn1
  T_170066302__/RConn2 -- L_170066302/LConn2
  L_170066302/LConn3 -- T_170066302__/RConn3 -- bus520/LConn1
  T_239698383__/RConn1 -- L_239698383/LConn1
  T_239698383__/RConn2 -- L_239698383/LConn2
  L_239698383/LConn3 -- T_239698383__/RConn3 -- bus521/LConn1
  T_167924823__/RConn1 -- L_167924823/LConn1
  T_167924823__/RConn2 -- L_167924823/LConn2
  L_167924823/LConn3 -- T_167924823__/RConn3 -- bus522/LConn1
  T_224939099__Kewdale_sub_station/RConn1 -- L_224939099/LConn1
  T_224939099__Kewdale_sub_station/RConn2 -- L_224939099/LConn2
  L_224939099/LConn3 -- T_224939099__Kewdale_sub_station/RConn3 -- bus523/LConn1
  T_224958207__Belmont_sub_station/RConn1 -- L_224958207/LConn1
  T_224958207__Belmont_sub_station/RConn2 -- L_224958207/LConn2
  L_224958207/LConn3 -- T_224958207__Belmont_sub_station/RConn3 -- bus524/LConn1
  T_165170273__/RConn1 -- L_165170273/LConn1
  T_165170273__/RConn2 -- L_165170273/LConn2
  L_165170273/LConn3 -- T_165170273__/RConn3 -- bus525/LConn1
  T_165169360__/RConn1 -- L_165169360/LConn1
  T_165169360__/RConn2 -- L_165169360/LConn2
  L_165169360/LConn3 -- T_165169360__/RConn3 -- bus526/LConn1
  T_171582050__Mooloolaba_Substation/RConn1 -- L_171582050/LConn1
  T_171582050__Mooloolaba_Substation/RConn2 -- L_171582050/LConn2
  L_171582050/LConn3 -- T_171582050__Mooloolaba_Substation/RConn3 -- bus527/LConn1
  T_170840487__Palmwoods_Substation/RConn1 -- L_170840487/LConn1
  T_170840487__Palmwoods_Substation/RConn2 -- L_170840487/LConn2
  L_170840487/LConn3 -- T_170840487__Palmwoods_Substation/RConn3 -- bus528/LConn1
  T_328503276__Alexandra_Headlands_Substation/RConn1 -- L_328503276/LConn1
  T_328503276__Alexandra_Headlands_Substation/RConn2 -- L_328503276/LConn2
  L_328503276/LConn3 -- T_328503276__Alexandra_Headlands_Substation/RConn3 -- bus529/LConn1
  T_164682851__/RConn1 -- L_164682851/LConn1
  T_164682851__/RConn2 -- L_164682851/LConn2
  L_164682851/LConn3 -- T_164682851__/RConn3 -- bus530/LConn1
  T_192518673__Craiglie_132kV_Substation/RConn1 -- L_192518673/LConn1
  T_192518673__Craiglie_132kV_Substation/RConn2 -- L_192518673/LConn2
  L_192518673/LConn3 -- T_192518673__Craiglie_132kV_Substation/RConn3 -- bus531/LConn1
  T_171735144__/RConn1 -- L_171735144/LConn1
  T_171735144__/RConn2 -- L_171735144/LConn2
  L_171735144/LConn3 -- T_171735144__/RConn3 -- bus532/LConn1
  T_173551375__Isis_substation/RConn1 -- L_173551375/LConn1
  T_173551375__Isis_substation/RConn2 -- L_173551375/LConn2
  L_173551375/LConn3 -- T_173551375__Isis_substation/RConn3 -- bus533/LConn1
  T_171734315__Kilkivan_Substation/RConn1 -- L_171734315/LConn1
  T_171734315__Kilkivan_Substation/RConn2 -- L_171734315/LConn2
  L_171734315/LConn3 -- T_171734315__Kilkivan_Substation/RConn3 -- bus534/LConn1
  T_45727591__/RConn1 -- L_45727591/LConn1
  T_45727591__/RConn2 -- L_45727591/LConn2
  L_45727591/LConn3 -- T_45727591__/RConn3 -- bus535/LConn1
  T_439689405_132000_Cooma/RConn1 -- L_439689405/LConn1
  T_439689405_132000_Cooma/RConn2 -- L_439689405/LConn2
  L_439689405/LConn3 -- T_439689405_132000_Cooma/RConn3 -- bus536/LConn1
  T_121671797__Transgrid_Port_Macquarie_Substation/RConn1 -- L_121671797/LConn1
  T_121671797__Transgrid_Port_Macquarie_Substation/RConn2 -- L_121671797/LConn2
  L_121671797/LConn3 -- T_121671797__Transgrid_Port_Macquarie_Substation/RConn3 -- bus537/LConn1
  T_205011577_132000_Kempsey_subtransmission_substation/RConn1 -- L_205011577/LConn1
  T_205011577_132000_Kempsey_subtransmission_substation/RConn2 -- L_205011577/LConn2
  L_205011577/LConn3 -- T_205011577_132000_Kempsey_subtransmission_substation/RConn3 -- bus538/LConn1
  T_312551544__/RConn1 -- L_312551544/LConn1
  T_312551544__/RConn2 -- L_312551544/LConn2
  L_312551544/LConn3 -- T_312551544__/RConn3 -- bus539/LConn1
  T_69034090__/RConn1 -- L_69034090/LConn1
  T_69034090__/RConn2 -- L_69034090/LConn2
  L_69034090/LConn3 -- T_69034090__/RConn3 -- bus540/LConn1
  T_254440062__/RConn1 -- L_254440062/LConn1
  T_254440062__/RConn2 -- L_254440062/LConn2
  L_254440062/LConn3 -- T_254440062__/RConn3 -- bus541/LConn1
  T_161829167__Ourimbah_Substation/RConn1 -- L_161829167/LConn1
  T_161829167__Ourimbah_Substation/RConn2 -- L_161829167/LConn2
  L_161829167/LConn3 -- T_161829167__Ourimbah_Substation/RConn3 -- bus542/LConn1
  T_165712061__/RConn1 -- L_165712061/LConn1
  T_165712061__/RConn2 -- L_165712061/LConn2
  L_165712061/LConn3 -- T_165712061__/RConn3 -- bus543/LConn1
  T_179068556__Hornsby_Substation/RConn1 -- L_179068556/LConn1
  T_179068556__Hornsby_Substation/RConn2 -- L_179068556/LConn2
  L_179068556/LConn3 -- T_179068556__Hornsby_Substation/RConn3 -- bus544/LConn1
  T_178929982__/RConn1 -- L_178929982/LConn1
  T_178929982__/RConn2 -- L_178929982/LConn2
  L_178929982/LConn3 -- T_178929982__/RConn3 -- bus545/LConn1
  T_179085999__/RConn1 -- L_179085999/LConn1
  T_179085999__/RConn2 -- L_179085999/LConn2
  L_179085999/LConn3 -- T_179085999__/RConn3 -- bus546/LConn1
  T_50334999__Transgrid_Mulwala_Substation/RConn1 -- L_50334999/LConn1
  T_50334999__Transgrid_Mulwala_Substation/RConn2 -- L_50334999/LConn2
  L_50334999/LConn3 -- T_50334999__Transgrid_Mulwala_Substation/RConn3 -- bus547/LConn1
  T_108712269__/RConn1 -- L_108712269/LConn1
  T_108712269__/RConn2 -- L_108712269/LConn2
  L_108712269/LConn3 -- T_108712269__/RConn3 -- bus548/LConn1
  T_255998100_132000;33000_Mount_Terry_Transmission_Substation/RConn1 -- L_255998100/LConn1
  T_255998100_132000;33000_Mount_Terry_Transmission_Substation/RConn2 -- L_255998100/LConn2
  L_255998100/LConn3 -- T_255998100_132000;33000_Mount_Terry_Transmission_Substation/RConn3 -- bus549/LConn1
  T_239285915__/RConn1 -- L_239285915/LConn1
  T_239285915__/RConn2 -- L_239285915/LConn2
  L_239285915/LConn3 -- T_239285915__/RConn3 -- bus550/LConn1
  T_166089888__Beresfield_Substransmission_Substation/RConn1 -- L_166089888/LConn1
  T_166089888__Beresfield_Substransmission_Substation/RConn2 -- L_166089888/LConn2
  L_166089888/LConn3 -- T_166089888__Beresfield_Substransmission_Substation/RConn3 -- bus551/LConn1
  T_255998114__BOC_Substation/RConn1 -- L_255998114/LConn1
  T_255998114__BOC_Substation/RConn2 -- L_255998114/LConn2
  L_255998114/LConn3 -- T_255998114__BOC_Substation/RConn3 -- bus552/LConn1
  T_142733661_132000;33000_Springhill_Transmission_Substation/RConn1 -- L_142733661/LConn1
  T_142733661_132000;33000_Springhill_Transmission_Substation/RConn2 -- L_142733661/LConn2
  L_142733661/LConn3 -- T_142733661_132000;33000_Springhill_Transmission_Substation/RConn3 -- bus553/LConn1
  T_174246471__/RConn1 -- L_174246471/LConn1
  T_174246471__/RConn2 -- L_174246471/LConn2
  L_174246471/LConn3 -- T_174246471__/RConn3 -- bus554/LConn1
  T_363077936_132000_/RConn1 -- L_363077936/LConn1
  T_363077936_132000_/RConn2 -- L_363077936/LConn2
  L_363077936/LConn3 -- T_363077936_132000_/RConn3 -- bus555/LConn1
  T_174246481__/RConn1 -- L_174246481/LConn1
  T_174246481__/RConn2 -- L_174246481/LConn2
  L_174246481/LConn3 -- T_174246481__/RConn3 -- bus556/LConn1
  T_180773850__/RConn1 -- L_180773850/LConn1
  T_180773850__/RConn2 -- L_180773850/LConn2
  L_180773850/LConn3 -- T_180773850__/RConn3 -- bus557/LConn1
  T_267376696_132000;33000_Fairfax_Lane_Transmission_Substation/RConn1 -- L_267376696/LConn1
  T_267376696_132000;33000_Fairfax_Lane_Transmission_Substation/RConn2 -- L_267376696/LConn2
  L_267376696/LConn3 -- T_267376696_132000;33000_Fairfax_Lane_Transmission_Substation/RConn3 -- bus558/LConn1
  T_170407602__/RConn1 -- L_170407602/LConn1
  T_170407602__/RConn2 -- L_170407602/LConn2
  L_170407602/LConn3 -- T_170407602__/RConn3 -- bus559/LConn1
  T_170407657__/RConn1 -- L_170407657/LConn1
  T_170407657__/RConn2 -- L_170407657/LConn2
  L_170407657/LConn3 -- T_170407657__/RConn3 -- bus560/LConn1
  T_173401274__/RConn1 -- L_173401274/LConn1
  T_173401274__/RConn2 -- L_173401274/LConn2
  L_173401274/LConn3 -- T_173401274__/RConn3 -- bus561/LConn1
  T_174991765__/RConn1 -- L_174991765/LConn1
  T_174991765__/RConn2 -- L_174991765/LConn2
  L_174991765/LConn3 -- T_174991765__/RConn3 -- bus562/LConn1
  T_83991232__/RConn1 -- L_83991232/LConn1
  T_83991232__/RConn2 -- L_83991232/LConn2
  L_83991232/LConn3 -- T_83991232__/RConn3 -- bus563/LConn1
  T_174239045__/RConn1 -- L_174239045/LConn1
  T_174239045__/RConn2 -- L_174239045/LConn2
  L_174239045/LConn3 -- T_174239045__/RConn3 -- bus564/LConn1
  T_172245698__/RConn1 -- L_172245698/LConn1
  T_172245698__/RConn2 -- L_172245698/LConn2
  L_172245698/LConn3 -- T_172245698__/RConn3 -- bus565/LConn1
  T_171845369__/RConn1 -- L_171845369/LConn1
  T_171845369__/RConn2 -- L_171845369/LConn2
  L_171845369/LConn3 -- T_171845369__/RConn3 -- bus566/LConn1
  T_172246489__/RConn1 -- L_172246489/LConn1
  T_172246489__/RConn2 -- L_172246489/LConn2
  L_172246489/LConn3 -- T_172246489__/RConn3 -- bus567/LConn1
  T_242555644__/RConn1 -- L_242555644/LConn1
  T_242555644__/RConn2 -- L_242555644/LConn2
  L_242555644/LConn3 -- T_242555644__/RConn3 -- bus568/LConn1
  T_164774384__/RConn1 -- L_164774384/LConn1
  T_164774384__/RConn2 -- L_164774384/LConn2
  L_164774384/LConn3 -- T_164774384__/RConn3 -- bus569/LConn1
  T_234528471__/RConn1 -- L_234528471/LConn1
  T_234528471__/RConn2 -- L_234528471/LConn2
  L_234528471/LConn3 -- T_234528471__/RConn3 -- bus570/LConn1
  T_164025782__/RConn1 -- L_164025782/LConn1
  T_164025782__/RConn2 -- L_164025782/LConn2
  L_164025782/LConn3 -- T_164025782__/RConn3 -- bus571/LConn1
  T_196583887_132000_132_kV_Kareeya/RConn1 -- L_196583887/LConn1
  T_196583887_132000_132_kV_Kareeya/RConn2 -- L_196583887/LConn2
  L_196583887/LConn3 -- T_196583887_132000_132_kV_Kareeya/RConn3 -- bus572/LConn1
  T_172998381__/RConn1 -- L_172998381/LConn1
  T_172998381__/RConn2 -- L_172998381/LConn2
  L_172998381/LConn3 -- T_172998381__/RConn3 -- bus573/LConn1
  T_298020591__/RConn1 -- L_298020591/LConn1
  T_298020591__/RConn2 -- L_298020591/LConn2
  L_298020591/LConn3 -- T_298020591__/RConn3 -- bus574/LConn1
  T_255775145_132000_Tallawarra_Substation/RConn1 -- L_255775145/LConn1
  T_255775145_132000_Tallawarra_Substation/RConn2 -- L_255775145/LConn2
  L_255775145/LConn3 -- T_255775145_132000_Tallawarra_Substation/RConn3 -- bus575/LConn1
  T_227898159_132000;33000_Bellambi_Transmission_Substation/RConn1 -- L_227898159/LConn1
  T_227898159_132000;33000_Bellambi_Transmission_Substation/RConn2 -- L_227898159/LConn2
  L_227898159/LConn3 -- T_227898159_132000;33000_Bellambi_Transmission_Substation/RConn3 -- bus576/LConn1
  T_224945355__/RConn1 -- L_224945355/LConn1
  T_224945355__/RConn2 -- L_224945355/LConn2
  L_224945355/LConn3 -- T_224945355__/RConn3 -- bus577/LConn1
  T_225196539__/RConn1 -- L_225196539/LConn1
  T_225196539__/RConn2 -- L_225196539/LConn2
  L_225196539/LConn3 -- T_225196539__/RConn3 -- bus578/LConn1
  T_171581252__/RConn1 -- L_171581252/LConn1
  T_171581252__/RConn2 -- L_171581252/LConn2
  L_171581252/LConn3 -- T_171581252__/RConn3 -- bus579/LConn1
  T_175017770__Bundaberg_substation/RConn1 -- L_175017770/LConn1
  T_175017770__Bundaberg_substation/RConn2 -- L_175017770/LConn2
  L_175017770/LConn3 -- T_175017770__Bundaberg_substation/RConn3 -- bus580/LConn1
  T_163374875__Latham_Substation/RConn1 -- L_163374875/LConn1
  T_163374875__Latham_Substation/RConn2 -- L_163374875/LConn2
  L_163374875/LConn3 -- T_163374875__Latham_Substation/RConn3 -- bus581/LConn1
  T_163374879__Belconnen_Substation/RConn1 -- L_163374879/LConn1
  T_163374879__Belconnen_Substation/RConn2 -- L_163374879/LConn2
  L_163374879/LConn3 -- T_163374879__Belconnen_Substation/RConn3 -- bus582/LConn1
  T_163374877__Gold_Creek_Substation/RConn1 -- L_163374877/LConn1
  T_163374877__Gold_Creek_Substation/RConn2 -- L_163374877/LConn2
  L_163374877/LConn3 -- T_163374877__Gold_Creek_Substation/RConn3 -- bus583/LConn1
  T_166184400__/RConn1 -- L_166184400/LConn1
  T_166184400__/RConn2 -- L_166184400/LConn2
  L_166184400/LConn3 -- T_166184400__/RConn3 -- bus584/LConn1
  T_171573029__Biloela_Substation/RConn1 -- L_171573029/LConn1
  T_171573029__Biloela_Substation/RConn2 -- L_171573029/LConn2
  L_171573029/LConn3 -- T_171573029__Biloela_Substation/RConn3 -- bus585/LConn1
  T_175020086__QR_Clayton_substation/RConn1 -- L_175020086/LConn1
  T_175020086__QR_Clayton_substation/RConn2 -- L_175020086/LConn2
  L_175020086/LConn3 -- T_175020086__QR_Clayton_substation/RConn3 -- bus586/LConn1
  T_165709781__/RConn1 -- L_165709781/LConn1
  T_165709781__/RConn2 -- L_165709781/LConn2
  L_165709781/LConn3 -- T_165709781__/RConn3 -- bus587/LConn1
  T_377141169__Charmhaven_Zone_Substation/RConn1 -- L_377141169/LConn1
  T_377141169__Charmhaven_Zone_Substation/RConn2 -- L_377141169/LConn2
  L_377141169/LConn3 -- T_377141169__Charmhaven_Zone_Substation/RConn3 -- bus588/LConn1
  T_218450415__/RConn1 -- L_218450415/LConn1
  T_218450415__/RConn2 -- L_218450415/LConn2
  L_218450415/LConn3 -- T_218450415__/RConn3 -- bus589/LConn1
  T_72231242__/RConn1 -- L_72231242/LConn1
  T_72231242__/RConn2 -- L_72231242/LConn2
  L_72231242/LConn3 -- T_72231242__/RConn3 -- bus590/LConn1
  T_171581834__/RConn1 -- L_171581834/LConn1
  T_171581834__/RConn2 -- L_171581834/LConn2
  L_171581834/LConn3 -- T_171581834__/RConn3 -- bus591/LConn1
  T_171846476__/RConn1 -- L_171846476/LConn1
  T_171846476__/RConn2 -- L_171846476/LConn2
  L_171846476/LConn3 -- T_171846476__/RConn3 -- bus592/LConn1
  T_166113109__/RConn1 -- L_166113109/LConn1
  T_166113109__/RConn2 -- L_166113109/LConn2
  L_166113109/LConn3 -- T_166113109__/RConn3 -- bus593/LConn1
  T_219209922__/RConn1 -- L_219209922/LConn1
  T_219209922__/RConn2 -- L_219209922/LConn2
  L_219209922/LConn3 -- T_219209922__/RConn3 -- bus594/LConn1
  T_255775138_132000;33000_Outer_Harbour_Transmission_Substation/RConn1 -- L_255775138/LConn1
  T_255775138_132000;33000_Outer_Harbour_Transmission_Substation/RConn2 -- L_255775138/LConn2
  L_255775138/LConn3 -- T_255775138_132000;33000_Outer_Harbour_Transmission_Substation/RConn3 -- bus595/LConn1
  T_46503657__Beechboro_Substation/RConn1 -- L_46503657/LConn1
  T_46503657__Beechboro_Substation/RConn2 -- L_46503657/LConn2
  L_46503657/LConn3 -- T_46503657__Beechboro_Substation/RConn3 -- bus596/LConn1
  T_171980651__/RConn1 -- L_171980651/LConn1
  T_171980651__/RConn2 -- L_171980651/LConn2
  L_171980651/LConn3 -- T_171980651__/RConn3 -- bus597/LConn1
  T_171189093__/RConn1 -- L_171189093/LConn1
  T_171189093__/RConn2 -- L_171189093/LConn2
  L_171189093/LConn3 -- T_171189093__/RConn3 -- bus598/LConn1
  T_328487572__Birtinya_Substation/RConn1 -- L_328487572/LConn1
  T_328487572__Birtinya_Substation/RConn2 -- L_328487572/LConn2
  L_328487572/LConn3 -- T_328487572__Birtinya_Substation/RConn3 -- bus599/LConn1
  T_328487570__Kawana_Substation/RConn1 -- L_328487570/LConn1
  T_328487570__Kawana_Substation/RConn2 -- L_328487570/LConn2
  L_328487570/LConn3 -- T_328487570__Kawana_Substation/RConn3 -- bus600/LConn1
  T_373381185__Hume_Streets_Sub_Station/RConn1 -- L_373381185/LConn1
  T_373381185__Hume_Streets_Sub_Station/RConn2 -- L_373381185/LConn2
  L_373381185/LConn3 -- T_373381185__Hume_Streets_Sub_Station/RConn3 -- bus601/LConn1
  T_171979185__/RConn1 -- L_171979185/LConn1
  T_171979185__/RConn2 -- L_171979185/LConn2
  L_171979185/LConn3 -- T_171979185__/RConn3 -- bus602/LConn1
  T_284934380__/RConn1 -- L_284934380/LConn1
  T_284934380__/RConn2 -- L_284934380/LConn2
  L_284934380/LConn3 -- T_284934380__/RConn3 -- bus603/LConn1
  T_259142988__/RConn1 -- L_259142988/LConn1
  T_259142988__/RConn2 -- L_259142988/LConn2
  L_259142988/LConn3 -- T_259142988__/RConn3 -- bus604/LConn1
  T_229813242__/RConn1 -- L_229813242/LConn1
  T_229813242__/RConn2 -- L_229813242/LConn2
  L_229813242/LConn3 -- T_229813242__/RConn3 -- bus605/LConn1
  T_229813239__/RConn1 -- L_229813239/LConn1
  T_229813239__/RConn2 -- L_229813239/LConn2
  L_229813239/LConn3 -- T_229813239__/RConn3 -- bus606/LConn1
  T_223942734__/RConn1 -- L_223942734/LConn1
  T_223942734__/RConn2 -- L_223942734/LConn2
  L_223942734/LConn3 -- T_223942734__/RConn3 -- bus607/LConn1
  T_346232962__TOA_Elaine_Terminal_Station/RConn1 -- L_346232962/LConn1
  T_346232962__TOA_Elaine_Terminal_Station/RConn2 -- L_346232962/LConn2
  L_346232962/LConn3 -- T_346232962__TOA_Elaine_Terminal_Station/RConn3 -- bus608/LConn1
  T_89180086__AusNet_Ballarat_Terminal_Station/RConn1 -- L_89180086/LConn1
  T_89180086__AusNet_Ballarat_Terminal_Station/RConn2 -- L_89180086/LConn2
  L_89180086/LConn3 -- T_89180086__AusNet_Ballarat_Terminal_Station/RConn3 -- bus609/LConn1
  T_104719368__George_Town_Substation/RConn1 -- L_104719368/LConn1
  T_104719368__George_Town_Substation/RConn2 -- L_104719368/LConn2
  L_104719368/LConn3 -- T_104719368__George_Town_Substation/RConn3 -- bus610/LConn1
  T_107265156__/RConn1 -- L_107265156/LConn1
  T_107265156__/RConn2 -- L_107265156/LConn2
  L_107265156/LConn3 -- T_107265156__/RConn3 -- bus611/LConn1
  T_56234037__Eildon_Terminal_Station/RConn1 -- L_56234037/LConn1
  T_56234037__Eildon_Terminal_Station/RConn2 -- L_56234037/LConn2
  L_56234037/LConn3 -- T_56234037__Eildon_Terminal_Station/RConn3 -- bus612/LConn1
  T_193910534__/RConn1 -- L_193910534/LConn1
  T_193910534__/RConn2 -- L_193910534/LConn2
  L_193910534/LConn3 -- T_193910534__/RConn3 -- bus613/LConn1
  T_156598151__AusNet_Terang_Terminal_Station/RConn1 -- L_156598151/LConn1
  T_156598151__AusNet_Terang_Terminal_Station/RConn2 -- L_156598151/LConn2
  L_156598151/LConn3 -- T_156598151__AusNet_Terang_Terminal_Station/RConn3 -- bus614/LConn1
  T_104720150__Basslink_DC_AC_convertor_station/RConn1 -- L_104720150/LConn1
  T_104720150__Basslink_DC_AC_convertor_station/RConn2 -- L_104720150/LConn2
  L_104720150/LConn3 -- T_104720150__Basslink_DC_AC_convertor_station/RConn3 -- bus615/LConn1
  T_235143897__SP_AusNet_Brooklyn_Terminal_Station/RConn1 -- L_235143897/LConn1
  T_235143897__SP_AusNet_Brooklyn_Terminal_Station/RConn2 -- L_235143897/LConn2
  L_235143897/LConn3 -- T_235143897__SP_AusNet_Brooklyn_Terminal_Station/RConn3 -- bus616/LConn1
  T_384601555__AusNet_Fishermans_Bend_Terminal_Station/RConn1 -- L_384601555/LConn1
  T_384601555__AusNet_Fishermans_Bend_Terminal_Station/RConn2 -- L_384601555/LConn2
  L_384601555/LConn3 -- T_384601555__AusNet_Fishermans_Bend_Terminal_Station/RConn3 -- bus617/LConn1
  T_28225387__SP_AusNet_Malvern_Terminal_Station/RConn1 -- L_28225387/LConn1
  T_28225387__SP_AusNet_Malvern_Terminal_Station/RConn2 -- L_28225387/LConn2
  L_28225387/LConn3 -- T_28225387__SP_AusNet_Malvern_Terminal_Station/RConn3 -- bus618/LConn1
  T_239972088__SP_AusNet_Rowville_East_Terminal_Station/RConn1 -- L_239972088/LConn1
  T_239972088__SP_AusNet_Rowville_East_Terminal_Station/RConn2 -- L_239972088/LConn2
  L_239972088/LConn3 -- T_239972088__SP_AusNet_Rowville_East_Terminal_Station/RConn3 -- bus619/LConn1
  T_30837800__SP_AusNet_Richmond_Terminal_Station/RConn1 -- L_30837800/LConn1
  T_30837800__SP_AusNet_Richmond_Terminal_Station/RConn2 -- L_30837800/LConn2
  L_30837800/LConn3 -- T_30837800__SP_AusNet_Richmond_Terminal_Station/RConn3 -- bus620/LConn1
  T_134534513__AusNet_Springvale_Terminal_Station/RConn1 -- L_134534513/LConn1
  T_134534513__AusNet_Springvale_Terminal_Station/RConn2 -- L_134534513/LConn2
  L_134534513/LConn3 -- T_134534513__AusNet_Springvale_Terminal_Station/RConn3 -- bus621/LConn1
  T_169794711__/RConn1 -- L_169794711/LConn1
  T_169794711__/RConn2 -- L_169794711/LConn2
  L_169794711/LConn3 -- T_169794711__/RConn3 -- bus622/LConn1
  T_172740336__/RConn1 -- L_172740336/LConn1
  T_172740336__/RConn2 -- L_172740336/LConn2
  L_172740336/LConn3 -- T_172740336__/RConn3 -- bus623/LConn1
  T_41098451_220000;22000_SP_AusNet_Brunswick_Terminal_Station/RConn1 -- L_41098451/LConn1
  T_41098451_220000;22000_SP_AusNet_Brunswick_Terminal_Station/RConn2 -- L_41098451/LConn2
  L_41098451/LConn3 -- T_41098451_220000;22000_SP_AusNet_Brunswick_Terminal_Station/RConn3 -- bus624/LConn1
  T_24577195__SP_AusNet_Ringwood_Terminal_Station/RConn1 -- L_24577195/LConn1
  T_24577195__SP_AusNet_Ringwood_Terminal_Station/RConn2 -- L_24577195/LConn2
  L_24577195/LConn3 -- T_24577195__SP_AusNet_Ringwood_Terminal_Station/RConn3 -- bus625/LConn1
  T_23718111__SP_AusNet_Templestowe_Terminal_Station/RConn1 -- L_23718111/LConn1
  T_23718111__SP_AusNet_Templestowe_Terminal_Station/RConn2 -- L_23718111/LConn2
  L_23718111/LConn3 -- T_23718111__SP_AusNet_Templestowe_Terminal_Station/RConn3 -- bus626/LConn1
  T_244141232__SP_AusNet_Geelong_Terminal_Station/RConn1 -- L_244141232/LConn1
  T_244141232__SP_AusNet_Geelong_Terminal_Station/RConn2 -- L_244141232/LConn2
  L_244141232/LConn3 -- T_244141232__SP_AusNet_Geelong_Terminal_Station/RConn3 -- bus627/LConn1
  T_169793928__/RConn1 -- L_169793928/LConn1
  T_169793928__/RConn2 -- L_169793928/LConn2
  L_169793928/LConn3 -- T_169793928__/RConn3 -- bus628/LConn1
  T_239996090__SP_AusNet_Wemen_Terminal_Station/RConn1 -- L_239996090/LConn1
  T_239996090__SP_AusNet_Wemen_Terminal_Station/RConn2 -- L_239996090/LConn2
  L_239996090/LConn3 -- T_239996090__SP_AusNet_Wemen_Terminal_Station/RConn3 -- bus629/LConn1
  T_64943050__SP_AusNet_South_Morang_Terminal_Station/RConn1 -- L_64943050/LConn1
  T_64943050__SP_AusNet_South_Morang_Terminal_Station/RConn2 -- L_64943050/LConn2
  L_64943050/LConn3 -- T_64943050__SP_AusNet_South_Morang_Terminal_Station/RConn3 -- bus630/LConn1
  T_205163985__Glenrowan_Terminal_Station/RConn1 -- L_205163985/LConn1
  T_205163985__Glenrowan_Terminal_Station/RConn2 -- L_205163985/LConn2
  L_205163985/LConn3 -- T_205163985__Glenrowan_Terminal_Station/RConn3 -- bus631/LConn1
  T_23718970__SP_AusNet_Thomastown_Terminal_Station/RConn1 -- L_23718970/LConn1
  T_23718970__SP_AusNet_Thomastown_Terminal_Station/RConn2 -- L_23718970/LConn2
  L_23718970/LConn3 -- T_23718970__SP_AusNet_Thomastown_Terminal_Station/RConn3 -- bus632/LConn1
  T_87325631__/RConn1 -- L_87325631/LConn1
  T_87325631__/RConn2 -- L_87325631/LConn2
  L_87325631/LConn3 -- T_87325631__/RConn3 -- bus633/LConn1
  T_223940475__/RConn1 -- L_223940475/LConn1
  T_223940475__/RConn2 -- L_223940475/LConn2
  L_223940475/LConn3 -- T_223940475__/RConn3 -- bus634/LConn1
  T_28917073__SP_AusNet_Heatherton_Terminal_Station/RConn1 -- L_28917073/LConn1
  T_28917073__SP_AusNet_Heatherton_Terminal_Station/RConn2 -- L_28917073/LConn2
  L_28917073/LConn3 -- T_28917073__SP_AusNet_Heatherton_Terminal_Station/RConn3 -- bus635/LConn1
  T_218402190__/RConn1 -- L_218402190/LConn1
  T_218402190__/RConn2 -- L_218402190/LConn2
  L_218402190/LConn3 -- T_218402190__/RConn3 -- bus636/LConn1
  T_229759860__/RConn1 -- L_229759860/LConn1
  T_229759860__/RConn2 -- L_229759860/LConn2
  L_229759860/LConn3 -- T_229759860__/RConn3 -- bus637/LConn1
  T_174893662__Shepparton_Terminal_Station/RConn1 -- L_174893662/LConn1
  T_174893662__Shepparton_Terminal_Station/RConn2 -- L_174893662/LConn2
  L_174893662/LConn3 -- T_174893662__Shepparton_Terminal_Station/RConn3 -- bus638/LConn1
  T_173566563__AusNet_Foxterville_Terminal_Station/RConn1 -- L_173566563/LConn1
  T_173566563__AusNet_Foxterville_Terminal_Station/RConn2 -- L_173566563/LConn2
  L_173566563/LConn3 -- T_173566563__AusNet_Foxterville_Terminal_Station/RConn3 -- bus639/LConn1
  T_208198646__AusNet_West_Melbourne_Terminal_Station/RConn1 -- L_208198646/LConn1
  T_208198646__AusNet_West_Melbourne_Terminal_Station/RConn2 -- L_208198646/LConn2
  L_208198646/LConn3 -- T_208198646__AusNet_West_Melbourne_Terminal_Station/RConn3 -- bus640/LConn1
  T_223939702__/RConn1 -- L_223939702/LConn1
  T_223939702__/RConn2 -- L_223939702/LConn2
  L_223939702/LConn3 -- T_223939702__/RConn3 -- bus641/LConn1
  T_189021414__/RConn1 -- L_189021414/LConn1
  T_189021414__/RConn2 -- L_189021414/LConn2
  L_189021414/LConn3 -- T_189021414__/RConn3 -- bus642/LConn1
  T_172587651__Greenbank_Substation/RConn1 -- L_172587651/LConn1
  T_172587651__Greenbank_Substation/RConn2 -- L_172587651/LConn2
  L_172587651/LConn3 -- T_172587651__Greenbank_Substation/RConn3 -- bus643/LConn1
  T_176443359__Bundamba_Substation/RConn1 -- L_176443359/LConn1
  T_176443359__Bundamba_Substation/RConn2 -- L_176443359/LConn2
  L_176443359/LConn3 -- T_176443359__Bundamba_Substation/RConn3 -- bus644/LConn1
  T_173222725__/RConn1 -- L_173222725/LConn1
  T_173222725__/RConn2 -- L_173222725/LConn2
  L_173222725/LConn3 -- T_173222725__/RConn3 -- bus645/LConn1
  T_170709510__/RConn1 -- L_170709510/LConn1
  T_170709510__/RConn2 -- L_170709510/LConn2
  L_170709510/LConn3 -- T_170709510__/RConn3 -- bus646/LConn1
  T_170832455__/RConn1 -- L_170832455/LConn1
  T_170832455__/RConn2 -- L_170832455/LConn2
  L_170832455/LConn3 -- T_170832455__/RConn3 -- bus647/LConn1
  T_153737699__/RConn1 -- L_153737699/LConn1
  T_153737699__/RConn2 -- L_153737699/LConn2
  L_153737699/LConn3 -- T_153737699__/RConn3 -- bus648/LConn1
  T_171170697__/RConn1 -- L_171170697/LConn1
  T_171170697__/RConn2 -- L_171170697/LConn2
  L_171170697/LConn3 -- T_171170697__/RConn3 -- bus649/LConn1
  T_171728751__Gin_Gin_terminal_station/RConn1 -- L_171728751/LConn1
  T_171728751__Gin_Gin_terminal_station/RConn2 -- L_171728751/LConn2
  L_171728751/LConn3 -- T_171728751__Gin_Gin_terminal_station/RConn3 -- bus650/LConn1
  T_119995150__Callide_Switch_Yard/RConn1 -- L_119995150/LConn1
  T_119995150__Callide_Switch_Yard/RConn2 -- L_119995150/LConn2
  L_119995150/LConn3 -- T_119995150__Callide_Switch_Yard/RConn3 -- bus651/LConn1
  T_171486427__/RConn1 -- L_171486427/LConn1
  T_171486427__/RConn2 -- L_171486427/LConn2
  L_171486427/LConn3 -- T_171486427__/RConn3 -- bus652/LConn1
  T_172715843__Electranet_Northfield_Substation/RConn1 -- L_172715843/LConn1
  T_172715843__Electranet_Northfield_Substation/RConn2 -- L_172715843/LConn2
  L_172715843/LConn3 -- T_172715843__Electranet_Northfield_Substation/RConn3 -- bus653/LConn1
  T_169673123__Heywood/RConn1 -- L_169673123/LConn1
  T_169673123__Heywood/RConn2 -- L_169673123/LConn2
  L_169673123/LConn3 -- T_169673123__Heywood/RConn3 -- bus654/LConn1
  T_224209320__/RConn1 -- L_224209320/LConn1
  T_224209320__/RConn2 -- L_224209320/LConn2
  L_224209320/LConn3 -- T_224209320__/RConn3 -- bus655/LConn1
  T_172362099__/RConn1 -- L_172362099/LConn1
  T_172362099__/RConn2 -- L_172362099/LConn2
  L_172362099/LConn3 -- T_172362099__/RConn3 -- bus656/LConn1
  T_172364007__Cherry_Gardens_substation/RConn1 -- L_172364007/LConn1
  T_172364007__Cherry_Gardens_substation/RConn2 -- L_172364007/LConn2
  L_172364007/LConn3 -- T_172364007__Cherry_Gardens_substation/RConn3 -- bus657/LConn1
  T_170058930__/RConn1 -- L_170058930/LConn1
  T_170058930__/RConn2 -- L_170058930/LConn2
  L_170058930/LConn3 -- T_170058930__/RConn3 -- bus658/LConn1
  T_120511705__/RConn1 -- L_120511705/LConn1
  T_120511705__/RConn2 -- L_120511705/LConn2
  L_120511705/LConn3 -- T_120511705__/RConn3 -- bus659/LConn1
  T_170036971__/RConn1 -- L_170036971/LConn1
  T_170036971__/RConn2 -- L_170036971/LConn2
  L_170036971/LConn3 -- T_170036971__/RConn3 -- bus660/LConn1
  T_172714955__/RConn1 -- L_172714955/LConn1
  T_172714955__/RConn2 -- L_172714955/LConn2
  L_172714955/LConn3 -- T_172714955__/RConn3 -- bus661/LConn1
  T_173700961__/RConn1 -- L_173700961/LConn1
  T_173700961__/RConn2 -- L_173700961/LConn2
  L_173700961/LConn3 -- T_173700961__/RConn3 -- bus662/LConn1
  T_121646942__/RConn1 -- L_121646942/LConn1
  T_121646942__/RConn2 -- L_121646942/LConn2
  L_121646942/LConn3 -- T_121646942__/RConn3 -- bus663/LConn1
  T_172364006__Electranet_Magill_Substation/RConn1 -- L_172364006/LConn1
  T_172364006__Electranet_Magill_Substation/RConn2 -- L_172364006/LConn2
  L_172364006/LConn3 -- T_172364006__Electranet_Magill_Substation/RConn3 -- bus664/LConn1
  T_172867383__/RConn1 -- L_172867383/LConn1
  T_172867383__/RConn2 -- L_172867383/LConn2
  L_172867383/LConn3 -- T_172867383__/RConn3 -- bus665/LConn1
  T_204894935__/RConn1 -- L_204894935/LConn1
  T_204894935__/RConn2 -- L_204894935/LConn2
  L_204894935/LConn3 -- T_204894935__/RConn3 -- bus666/LConn1
  T_45237469__Sydney_West_Bulk_Supply_Point/RConn1 -- L_45237469/LConn1
  T_45237469__Sydney_West_Bulk_Supply_Point/RConn2 -- L_45237469/LConn2
  L_45237469/LConn3 -- T_45237469__Sydney_West_Bulk_Supply_Point/RConn3 -- bus667/LConn1
  T_376493893__Vales_Point_Substation/RConn1 -- L_376493893/LConn1
  T_376493893__Vales_Point_Substation/RConn2 -- L_376493893/LConn2
  L_376493893/LConn3 -- T_376493893__Vales_Point_Substation/RConn3 -- bus668/LConn1
  T_87853100__/RConn1 -- L_87853100/LConn1
  T_87853100__/RConn2 -- L_87853100/LConn2
  L_87853100/LConn3 -- T_87853100__/RConn3 -- bus669/LConn1
  T_194289858__Muja_Switchyard/RConn1 -- L_194289858/LConn1
  T_194289858__Muja_Switchyard/RConn2 -- L_194289858/LConn2
  L_194289858/LConn3 -- T_194289858__Muja_Switchyard/RConn3 -- bus670/LConn1
  T_223957157__/RConn1 -- L_223957157/LConn1
  T_223957157__/RConn2 -- L_223957157/LConn2
  L_223957157/LConn3 -- T_223957157__/RConn3 -- bus671/LConn1
  T_224223244__/RConn1 -- L_224223244/LConn1
  T_224223244__/RConn2 -- L_224223244/LConn2
  L_224223244/LConn3 -- T_224223244__/RConn3 -- bus672/LConn1
  T_172887193__Bulli_Creek_substation/RConn1 -- L_172887193/LConn1
  T_172887193__Bulli_Creek_substation/RConn2 -- L_172887193/LConn2
  L_172887193/LConn3 -- T_172887193__Bulli_Creek_substation/RConn3 -- bus673/LConn1
  T_168227360__/RConn1 -- L_168227360/LConn1
  T_168227360__/RConn2 -- L_168227360/LConn2
  L_168227360/LConn3 -- T_168227360__/RConn3 -- bus674/LConn1
  T_24038114__/RConn1 -- L_24038114/LConn1
  T_24038114__/RConn2 -- L_24038114/LConn2
  L_24038114/LConn3 -- T_24038114__/RConn3 -- bus675/LConn1
  T_172887491_330000_Dumaresq_switching_station/RConn1 -- L_172887491/LConn1
  T_172887491_330000_Dumaresq_switching_station/RConn2 -- L_172887491/LConn2
  L_172887491/LConn3 -- T_172887491_330000_Dumaresq_switching_station/RConn3 -- bus676/LConn1
  T_170833885__/RConn1 -- L_170833885/LConn1
  T_170833885__/RConn2 -- L_170833885/LConn2
  L_170833885/LConn3 -- T_170833885__/RConn3 -- bus677/LConn1
  T_173873963__Kemps_Creek/RConn1 -- L_173873963/LConn1
  T_173873963__Kemps_Creek/RConn2 -- L_173873963/LConn2
  L_173873963/LConn3 -- T_173873963__Kemps_Creek/RConn3 -- bus678/LConn1
  T_203043714__/RConn1 -- L_203043714/LConn1
  T_203043714__/RConn2 -- L_203043714/LConn2
  L_203043714/LConn3 -- T_203043714__/RConn3 -- bus679/LConn1
  T_172739944__Avon_Transmission_Substation/RConn1 -- L_172739944/LConn1
  T_172739944__Avon_Transmission_Substation/RConn2 -- L_172739944/LConn2
  L_172739944/LConn3 -- T_172739944__Avon_Transmission_Substation/RConn3 -- bus680/LConn1
  T_171853256__Coffs_Harbour_subtransmission_station/RConn1 -- L_171853256/LConn1
  T_171853256__Coffs_Harbour_subtransmission_station/RConn2 -- L_171853256/LConn2
  L_171853256/LConn3 -- T_171853256__Coffs_Harbour_subtransmission_station/RConn3 -- bus681/LConn1
  T_179898706__/RConn1 -- L_179898706/LConn1
  T_179898706__/RConn2 -- L_179898706/LConn2
  L_179898706/LConn3 -- T_179898706__/RConn3 -- bus682/LConn1
  T_172609354__/RConn1 -- L_172609354/LConn1
  T_172609354__/RConn2 -- L_172609354/LConn2
  L_172609354/LConn3 -- T_172609354__/RConn3 -- bus683/LConn1
  T_164280399__/RConn1 -- L_164280399/LConn1
  T_164280399__/RConn2 -- L_164280399/LConn2
  L_164280399/LConn3 -- T_164280399__/RConn3 -- bus684/LConn1
  T_23717060__/RConn1 -- L_23717060/LConn1
  T_23717060__/RConn2 -- L_23717060/LConn2
  L_23717060/LConn3 -- T_23717060__/RConn3 -- bus685/LConn1
  T_77998934__/RConn1 -- L_77998934/LConn1
  T_77998934__/RConn2 -- L_77998934/LConn2
  L_77998934/LConn3 -- T_77998934__/RConn3 -- bus686/LConn1
  T_37106533__/RConn1 -- L_37106533/LConn1
  T_37106533__/RConn2 -- L_37106533/LConn2
  L_37106533/LConn3 -- T_37106533__/RConn3 -- bus687/LConn1
  T_167694317__/RConn1 -- L_167694317/LConn1
  T_167694317__/RConn2 -- L_167694317/LConn2
  L_167694317/LConn3 -- T_167694317__/RConn3 -- bus688/LConn1
  T_312550977__AusNet_Tarrone_Terminal_Station/RConn1 -- L_312550977/LConn1
  T_312550977__AusNet_Tarrone_Terminal_Station/RConn2 -- L_312550977/LConn2
  L_312550977/LConn3 -- T_312550977__AusNet_Tarrone_Terminal_Station/RConn3 -- bus689/LConn1
  T_146581911__/RConn1 -- L_146581911/LConn1
  T_146581911__/RConn2 -- L_146581911/LConn2
  L_146581911/LConn3 -- T_146581911__/RConn3 -- bus690/LConn1
  T_146581916_500000_/RConn1 -- L_146581916/LConn1
  T_146581916_500000_/RConn2 -- L_146581916/LConn2
  L_146581916/LConn3 -- T_146581916_500000_/RConn3 -- bus691/LConn1
  T_146579820__Loy_Yang_HVDC_Converter/RConn1 -- L_146579820/LConn1
  T_146579820__Loy_Yang_HVDC_Converter/RConn2 -- L_146579820/LConn2
  L_146579820/LConn3 -- T_146579820__Loy_Yang_HVDC_Converter/RConn3 -- bus692/LConn1
  T_23717059__/RConn1 -- L_23717059/LConn1
  T_23717059__/RConn2 -- L_23717059/LConn2
  L_23717059/LConn3 -- T_23717059__/RConn3 -- bus693/LConn1
  T_23647798__SP_AusNet_Sydenham_Terminal_Station/RConn1 -- L_23647798/LConn1
  T_23647798__SP_AusNet_Sydenham_Terminal_Station/RConn2 -- L_23647798/LConn2
  L_23647798/LConn3 -- T_23647798__SP_AusNet_Sydenham_Terminal_Station/RConn3 -- bus694/LConn1
